simulink model "model"  (R2016a)
(part 4 of 4)

  220_kV_Połaniec___Chmielów_CN_199098053_220000_CN_191352746_220000/RConn1 -- "T_199098053_400000;220000;110000;15000_Stacja_elektroenergetyczna_\"Połaniec\"_400_220_110kV"/RConn1 -- 220_kV_Połaniec___Radkowice_CN_199098053_220000_CN_199098055_220000/RConn1 -- _CN_199098053_220000_CN_130207099_220000/LConn1 -- L_199098053/LConn1
  220_kV_Połaniec___Chmielów_CN_199098053_220000_CN_191352746_220000/RConn2 -- "T_199098053_400000;220000;110000;15000_Stacja_elektroenergetyczna_\"Połaniec\"_400_220_110kV"/RConn2 -- 220_kV_Połaniec___Radkowice_CN_199098053_220000_CN_199098055_220000/RConn2 -- _CN_199098053_220000_CN_130207099_220000/LConn2 -- L_199098053/LConn2
  220_kV_Połaniec___Chmielów_CN_199098053_220000_CN_191352746_220000/RConn3 -- "T_199098053_400000;220000;110000;15000_Stacja_elektroenergetyczna_\"Połaniec\"_400_220_110kV"/RConn3 -- 220_kV_Połaniec___Radkowice_CN_199098053_220000_CN_199098055_220000/RConn3 -- _CN_199098053_220000_CN_130207099_220000/LConn3 -- L_199098053/LConn3 -- bus86/LConn1
  _CN_199098053_220000_CN_130207099_220000/RConn1 -- G_130207099_Elektrownia_Połaniec/RConn1 -- _CN_199098053_400000_CN_130207099_220000/LConn1
  _CN_199098053_220000_CN_130207099_220000/RConn2 -- G_130207099_Elektrownia_Połaniec/RConn2 -- _CN_199098053_400000_CN_130207099_220000/LConn2
  _CN_199098053_220000_CN_130207099_220000/RConn3 -- G_130207099_Elektrownia_Połaniec/RConn3 -- _CN_199098053_400000_CN_130207099_220000/LConn3 -- bus87/LConn1
  _CN_254235846_220000_CN_189851841_220000/RConn1 -- "T_254235846_400000;110000_Stacja_elektroenergetyczna_\"Ostrowiec\"_400_110_kV"/RConn1 -- L_254235846/LConn1
  _CN_254235846_220000_CN_189851841_220000/RConn2 -- "T_254235846_400000;110000_Stacja_elektroenergetyczna_\"Ostrowiec\"_400_110_kV"/RConn2 -- L_254235846/LConn2
  _CN_254235846_220000_CN_189851841_220000/RConn3 -- "T_254235846_400000;110000_Stacja_elektroenergetyczna_\"Ostrowiec\"_400_110_kV"/RConn3 -- L_254235846/LConn3 -- bus88/LConn1
  T_179279860_220000;110000_Stacja_elektroenergetyczna_„Ząbkowice”_220_110_kV/LConn1 -- 220kV_Ząbkowice___Groszowice_CN_336990960_220000_CN_179279860_220000/RConn1
  T_179279860_220000;110000_Stacja_elektroenergetyczna_„Ząbkowice”_220_110_kV/LConn2 -- 220kV_Ząbkowice___Groszowice_CN_336990960_220000_CN_179279860_220000/RConn2
  220kV_Ząbkowice___Groszowice_CN_336990960_220000_CN_179279860_220000/RConn3 -- T_179279860_220000;110000_Stacja_elektroenergetyczna_„Ząbkowice”_220_110_kV/LConn3 -- bus89/LConn1
  220kV_Turów___Mikułowa_CN_111615226_220000_CN_90038401_220000/RConn1 -- G_90038401_Elektrownia_Turów/RConn1 -- 400kV_Turów___Mikułowa_CN_111615226_400000_CN_90038401_220000/LConn1
  220kV_Turów___Mikułowa_CN_111615226_220000_CN_90038401_220000/RConn2 -- G_90038401_Elektrownia_Turów/RConn2 -- 400kV_Turów___Mikułowa_CN_111615226_400000_CN_90038401_220000/LConn2
  220kV_Turów___Mikułowa_CN_111615226_220000_CN_90038401_220000/RConn3 -- G_90038401_Elektrownia_Turów/RConn3 -- 400kV_Turów___Mikułowa_CN_111615226_400000_CN_90038401_220000/LConn3 -- bus90/LConn1
  220kV_Joachimów___Huta_Częstochowa_CN_224727316_220000_CN_217899005_220000/LConn1 -- "T_224727316__Stacja_elektroenergetyczna_\"Huta_Częstochowa\"_220_110_kV"/LConn1 -- 220kV_Joachimów___Huta_Częstochowa_CN_224727316_220000_CN_66161634_220000/RConn1 -- 220kV_Joachimów___Huta_Częstochowa_CN_224727316_220000_CN_241842600_220000/RConn1
  220kV_Joachimów___Huta_Częstochowa_CN_224727316_220000_CN_217899005_220000/LConn2 -- "T_224727316__Stacja_elektroenergetyczna_\"Huta_Częstochowa\"_220_110_kV"/LConn2 -- 220kV_Joachimów___Huta_Częstochowa_CN_224727316_220000_CN_66161634_220000/RConn2 -- 220kV_Joachimów___Huta_Częstochowa_CN_224727316_220000_CN_241842600_220000/RConn2
  220kV_Joachimów___Huta_Częstochowa_CN_224727316_220000_CN_217899005_220000/LConn3 -- "T_224727316__Stacja_elektroenergetyczna_\"Huta_Częstochowa\"_220_110_kV"/LConn3 -- 220kV_Joachimów___Huta_Częstochowa_CN_224727316_220000_CN_66161634_220000/RConn3 -- 220kV_Joachimów___Huta_Częstochowa_CN_224727316_220000_CN_241842600_220000/RConn3 -- bus91/LConn1
  "T_217899005_220000;110000_Stacja_elektroenergetyczna_\"Wrzosowa\"_220_110_kV"/LConn1 -- 220kV_Joachimów___Huta_Częstochowa_CN_224727316_220000_CN_217899005_220000/RConn1
  "T_217899005_220000;110000_Stacja_elektroenergetyczna_\"Wrzosowa\"_220_110_kV"/LConn2 -- 220kV_Joachimów___Huta_Częstochowa_CN_224727316_220000_CN_217899005_220000/RConn2
  220kV_Joachimów___Huta_Częstochowa_CN_224727316_220000_CN_217899005_220000/RConn3 -- "T_217899005_220000;110000_Stacja_elektroenergetyczna_\"Wrzosowa\"_220_110_kV"/LConn3 -- bus92/LConn1
  220_kV_Dunowo___Żydowo_CN_178838661_220000_CN_175406958_220000/RConn1 -- "T_175406958_400000;220000;110000_Stacja_elektroenergetyczna_\"Dunowo\"_400_220_110_kV"/RConn1 -- L_175406958/LConn1
  220_kV_Dunowo___Żydowo_CN_178838661_220000_CN_175406958_220000/RConn2 -- "T_175406958_400000;220000;110000_Stacja_elektroenergetyczna_\"Dunowo\"_400_220_110_kV"/RConn2 -- L_175406958/LConn2
  220_kV_Dunowo___Żydowo_CN_178838661_220000_CN_175406958_220000/RConn3 -- "T_175406958_400000;220000;110000_Stacja_elektroenergetyczna_\"Dunowo\"_400_220_110_kV"/RConn3 -- L_175406958/LConn3 -- bus93/LConn1
  T_29098336_220000;110000_Stacja_elektroenergetyczna_„Piaseczno”_220_110_kV/LConn1 -- 220kV_Mory___Piaseczno_CN_29115701_220000_CN_29098336_220000/RConn1
  T_29098336_220000;110000_Stacja_elektroenergetyczna_„Piaseczno”_220_110_kV/LConn2 -- 220kV_Mory___Piaseczno_CN_29115701_220000_CN_29098336_220000/RConn2
  220kV_Mory___Piaseczno_CN_29115701_220000_CN_29098336_220000/RConn3 -- T_29098336_220000;110000_Stacja_elektroenergetyczna_„Piaseczno”_220_110_kV/LConn3 -- bus94/LConn1
  "T_255293400_220000;110000_Stacja_elektroenergetyczna_\"Bydgoszcz_Zachód\"_220_110_kV"/LConn1 -- 220kV_Jasiniec___Bydgoszcz_Zachód_CN_46235456_220000_CN_255293400_220000/RConn1
  "T_255293400_220000;110000_Stacja_elektroenergetyczna_\"Bydgoszcz_Zachód\"_220_110_kV"/LConn2 -- 220kV_Jasiniec___Bydgoszcz_Zachód_CN_46235456_220000_CN_255293400_220000/RConn2
  220kV_Jasiniec___Bydgoszcz_Zachód_CN_46235456_220000_CN_255293400_220000/RConn3 -- "T_255293400_220000;110000_Stacja_elektroenergetyczna_\"Bydgoszcz_Zachód\"_220_110_kV"/LConn3 -- bus95/LConn1
  220kV_Mokre___Chełm_CN_194903381_220000_CN_170368942_220000/RConn1 -- "T_194903381_220000;110000_Stacja_elektroenergetyczna_\"Chełm\"_220_110_kV"/LConn1 -- 220kV_Mokre___Chełm_CN_194903381_220000_CN_170249563_220000/RConn1
  220kV_Mokre___Chełm_CN_194903381_220000_CN_170368942_220000/RConn2 -- "T_194903381_220000;110000_Stacja_elektroenergetyczna_\"Chełm\"_220_110_kV"/LConn2 -- 220kV_Mokre___Chełm_CN_194903381_220000_CN_170249563_220000/RConn2
  220kV_Mokre___Chełm_CN_194903381_220000_CN_170368942_220000/RConn3 -- "T_194903381_220000;110000_Stacja_elektroenergetyczna_\"Chełm\"_220_110_kV"/LConn3 -- 220kV_Mokre___Chełm_CN_194903381_220000_CN_170249563_220000/RConn3 -- bus96/LConn1
  "G_221120858_Elektrociepłownia_\"Zielona_Góra\"_S_A_"/RConn1 -- 220kV_Leśniów___Zielona_Góra_CN_158232924_220000_CN_221120858_220000/RConn1
  "G_221120858_Elektrociepłownia_\"Zielona_Góra\"_S_A_"/RConn2 -- 220kV_Leśniów___Zielona_Góra_CN_158232924_220000_CN_221120858_220000/RConn2
  220kV_Leśniów___Zielona_Góra_CN_158232924_220000_CN_221120858_220000/RConn3 -- "G_221120858_Elektrociepłownia_\"Zielona_Góra\"_S_A_"/RConn3 -- bus97/LConn1
  _CN_39428977_220000_CN_35222596_220000/RConn1 -- G_35222596_Elektrownia_Dolna_Odra/RConn1 -- _CN_39428977_400000_CN_35222596_220000/LConn1
  _CN_39428977_220000_CN_35222596_220000/RConn2 -- G_35222596_Elektrownia_Dolna_Odra/RConn2 -- _CN_39428977_400000_CN_35222596_220000/LConn2
  _CN_39428977_220000_CN_35222596_220000/RConn3 -- G_35222596_Elektrownia_Dolna_Odra/RConn3 -- _CN_39428977_400000_CN_35222596_220000/LConn3 -- bus98/LConn1
  T_177493901__/LConn1 -- _CN_39428977_220000_CN_177493901_220000/RConn1
  T_177493901__/LConn2 -- _CN_39428977_220000_CN_177493901_220000/RConn2
  _CN_39428977_220000_CN_177493901_220000/RConn3 -- T_177493901__/LConn3 -- bus99/LConn1
  T_240806770__/LConn1 -- _CN_240806770_220000_CN_153838553_220000/RConn1
  T_240806770__/LConn2 -- _CN_240806770_220000_CN_153838553_220000/RConn2
  _CN_240806770_220000_CN_153838553_220000/RConn3 -- T_240806770__/LConn3 -- bus100/LConn1
  _CN_179138441_220000_CN_276291999_220000/RConn1 -- "T_276291999__Stacja_elektroenergetyczna_\"Świebodzice\"_400_kV"/RConn1 -- L_276291999/LConn1
  _CN_179138441_220000_CN_276291999_220000/RConn2 -- "T_276291999__Stacja_elektroenergetyczna_\"Świebodzice\"_400_kV"/RConn2 -- L_276291999/LConn2
  _CN_179138441_220000_CN_276291999_220000/RConn3 -- "T_276291999__Stacja_elektroenergetyczna_\"Świebodzice\"_400_kV"/RConn3 -- L_276291999/LConn3 -- bus101/LConn1
  "T_198635989_220000;110000;30000;15000_Stacja_elektroenergetyczna_\"Boguchwała\"_220_110_kV"/LConn1 -- 220_kV_Chmielów___Boguchwała_CN_191352746_220000_CN_198635989_220000/RConn1
  "T_198635989_220000;110000;30000;15000_Stacja_elektroenergetyczna_\"Boguchwała\"_220_110_kV"/LConn2 -- 220_kV_Chmielów___Boguchwała_CN_191352746_220000_CN_198635989_220000/RConn2
  220_kV_Chmielów___Boguchwała_CN_191352746_220000_CN_198635989_220000/RConn3 -- "T_198635989_220000;110000;30000;15000_Stacja_elektroenergetyczna_\"Boguchwała\"_220_110_kV"/LConn3 -- bus102/LConn1
  400kV_Dobrzeń___Pasikurowice_CN_255277953_400000_CN_79033485_400000/LConn1 -- "T_255277953_400000;110000_Stacja_elektroenergetyczna_\"Dobrzeń\"_400_110_kV"/LConn1 -- 400kV_Dobrzeń___Pasikurowice_CN_255277953_400000_CN_171917072_400000/LConn1 -- 400kV_Dobrzeń___Pasikurowice_CN_255277953_400000_CN_241842600_400000/LConn1 -- 400kV_Dobrzeń___Wielopole_CN_255277953_400000_CN_139452056_400000/LConn1
  400kV_Dobrzeń___Pasikurowice_CN_255277953_400000_CN_79033485_400000/LConn2 -- "T_255277953_400000;110000_Stacja_elektroenergetyczna_\"Dobrzeń\"_400_110_kV"/LConn2 -- 400kV_Dobrzeń___Pasikurowice_CN_255277953_400000_CN_171917072_400000/LConn2 -- 400kV_Dobrzeń___Pasikurowice_CN_255277953_400000_CN_241842600_400000/LConn2 -- 400kV_Dobrzeń___Wielopole_CN_255277953_400000_CN_139452056_400000/LConn2
  400kV_Dobrzeń___Pasikurowice_CN_255277953_400000_CN_79033485_400000/LConn3 -- "T_255277953_400000;110000_Stacja_elektroenergetyczna_\"Dobrzeń\"_400_110_kV"/LConn3 -- 400kV_Dobrzeń___Pasikurowice_CN_255277953_400000_CN_171917072_400000/LConn3 -- 400kV_Dobrzeń___Pasikurowice_CN_255277953_400000_CN_241842600_400000/LConn3 -- 400kV_Dobrzeń___Wielopole_CN_255277953_400000_CN_139452056_400000/LConn3 -- bus103/LConn1
  400kV_Dobrzeń___Pasikurowice_CN_255277953_400000_CN_79033485_400000/RConn1 -- T_79033485_400000;110000_Stacja_elektroenergetyczna_„Pasikurowice”_400_110_kV/LConn1 -- 400kV_Pasikurowice___Ostrów_CN_79033485_400000_CN_255293403_400000/LConn1 -- 400kV_Pasikurowice___Wrocław_CN_79033485_400000_CN_154510504_400000/LConn1 -- 400kV_Czarna___Pasikurowice_CN_79033485_400000_CN_154894455_400000/LConn1
  400kV_Dobrzeń___Pasikurowice_CN_255277953_400000_CN_79033485_400000/RConn2 -- T_79033485_400000;110000_Stacja_elektroenergetyczna_„Pasikurowice”_400_110_kV/LConn2 -- 400kV_Pasikurowice___Ostrów_CN_79033485_400000_CN_255293403_400000/LConn2 -- 400kV_Pasikurowice___Wrocław_CN_79033485_400000_CN_154510504_400000/LConn2 -- 400kV_Czarna___Pasikurowice_CN_79033485_400000_CN_154894455_400000/LConn2
  400kV_Dobrzeń___Pasikurowice_CN_255277953_400000_CN_79033485_400000/RConn3 -- T_79033485_400000;110000_Stacja_elektroenergetyczna_„Pasikurowice”_400_110_kV/LConn3 -- 400kV_Pasikurowice___Ostrów_CN_79033485_400000_CN_255293403_400000/LConn3 -- 400kV_Pasikurowice___Wrocław_CN_79033485_400000_CN_154510504_400000/LConn3 -- bus104/LConn1 -- 400kV_Czarna___Pasikurowice_CN_79033485_400000_CN_154894455_400000/LConn3
  400kV_Dobrzeń___Pasikurowice_CN_255277953_400000_CN_171917072_400000/RConn1 -- T_171917072_400000;110000_Stacja_elektroenergetyczna_„Trębaczew”_400_110_kV/LConn1 -- 400kV_Rogowiec___Trębaczew_CN_171917072_400000_CN_255293403_400000/LConn1 -- 400kV_Rogowiec___Trębaczew_CN_171917072_400000_CN_293484891_400000/LConn1
  400kV_Dobrzeń___Pasikurowice_CN_255277953_400000_CN_171917072_400000/RConn2 -- T_171917072_400000;110000_Stacja_elektroenergetyczna_„Trębaczew”_400_110_kV/LConn2 -- 400kV_Rogowiec___Trębaczew_CN_171917072_400000_CN_255293403_400000/LConn2 -- 400kV_Rogowiec___Trębaczew_CN_171917072_400000_CN_293484891_400000/LConn2
  400kV_Dobrzeń___Pasikurowice_CN_255277953_400000_CN_171917072_400000/RConn3 -- T_171917072_400000;110000_Stacja_elektroenergetyczna_„Trębaczew”_400_110_kV/LConn3 -- 400kV_Rogowiec___Trębaczew_CN_171917072_400000_CN_255293403_400000/LConn3 -- 400kV_Rogowiec___Trębaczew_CN_171917072_400000_CN_293484891_400000/LConn3 -- bus105/LConn1
  400kV_Dobrzeń___Pasikurowice_CN_255277953_400000_CN_241842600_400000/RConn1 -- T_241842600_400000;220000_Stacja_elektroenergetyczna_„Joachimów”_400_220_kV/LConn1 -- 400kV_Wielopole___Joachimów_CN_241842600_400000_CN_40946784_400000/LConn1 -- 400kV_Wielopole___Joachimów_CN_241842600_400000_CN_66161634_400000/LConn1 -- 400kV_Wielopole___Joachimów_CN_241842600_400000_CN_293489607_400000/LConn1 -- 400kV_Wielopole___Joachimów_CN_241842600_400000_CN_139452056_400000/LConn1 -- 400kV_Wielopole___Joachimów_CN_241842600_400000_CN_293484891_400000/LConn1
  400kV_Dobrzeń___Pasikurowice_CN_255277953_400000_CN_241842600_400000/RConn2 -- T_241842600_400000;220000_Stacja_elektroenergetyczna_„Joachimów”_400_220_kV/LConn2 -- 400kV_Wielopole___Joachimów_CN_241842600_400000_CN_40946784_400000/LConn2 -- 400kV_Wielopole___Joachimów_CN_241842600_400000_CN_66161634_400000/LConn2 -- 400kV_Wielopole___Joachimów_CN_241842600_400000_CN_293489607_400000/LConn2 -- 400kV_Wielopole___Joachimów_CN_241842600_400000_CN_139452056_400000/LConn2 -- 400kV_Wielopole___Joachimów_CN_241842600_400000_CN_293484891_400000/LConn2
  400kV_Dobrzeń___Pasikurowice_CN_255277953_400000_CN_241842600_400000/RConn3 -- T_241842600_400000;220000_Stacja_elektroenergetyczna_„Joachimów”_400_220_kV/LConn3 -- 400kV_Wielopole___Joachimów_CN_241842600_400000_CN_40946784_400000/LConn3 -- 400kV_Wielopole___Joachimów_CN_241842600_400000_CN_66161634_400000/LConn3 -- 400kV_Wielopole___Joachimów_CN_241842600_400000_CN_293489607_400000/LConn3 -- 400kV_Wielopole___Joachimów_CN_241842600_400000_CN_139452056_400000/LConn3 -- 400kV_Wielopole___Joachimów_CN_241842600_400000_CN_293484891_400000/LConn3 -- bus106/LConn1
  400kV_Dobrzeń___Wielopole_CN_255277953_400000_CN_139452056_400000/RConn1 -- T_139452056_400000;220000;110000_Stacja_elektroenergetyczna_„Wielopole”_400_220_110_kV/LConn1 -- 400kV_Wielopole___Joachimów_CN_241842600_400000_CN_139452056_400000/RConn1
  400kV_Dobrzeń___Wielopole_CN_255277953_400000_CN_139452056_400000/RConn2 -- T_139452056_400000;220000;110000_Stacja_elektroenergetyczna_„Wielopole”_400_220_110_kV/LConn2 -- 400kV_Wielopole___Joachimów_CN_241842600_400000_CN_139452056_400000/RConn2
  400kV_Dobrzeń___Wielopole_CN_255277953_400000_CN_139452056_400000/RConn3 -- T_139452056_400000;220000;110000_Stacja_elektroenergetyczna_„Wielopole”_400_220_110_kV/LConn3 -- 400kV_Wielopole___Joachimów_CN_241842600_400000_CN_139452056_400000/RConn3 -- bus107/LConn1
  400kV_Wielopole___Joachimów_CN_241842600_400000_CN_40946784_400000/RConn1 -- T_40946784_400000;110000_Stacja_elektroenergetyczna_„Tucznawa”_400_110_kV/LConn1 -- 400_kV_Tarnów___Krosno_Iskrzynia_CN_166838338_400000_CN_40946784_400000/LConn1
  400kV_Wielopole___Joachimów_CN_241842600_400000_CN_40946784_400000/RConn2 -- T_40946784_400000;110000_Stacja_elektroenergetyczna_„Tucznawa”_400_110_kV/LConn2 -- 400_kV_Tarnów___Krosno_Iskrzynia_CN_166838338_400000_CN_40946784_400000/LConn2
  400kV_Wielopole___Joachimów_CN_241842600_400000_CN_40946784_400000/RConn3 -- T_40946784_400000;110000_Stacja_elektroenergetyczna_„Tucznawa”_400_110_kV/LConn3 -- 400_kV_Tarnów___Krosno_Iskrzynia_CN_166838338_400000_CN_40946784_400000/LConn3 -- bus108/LConn1
  "T_66161634_400000;220000;110000_Stacja_elektroenergetyczna_\"Łagisza\"_400_220_110_kV"/LConn1 -- 400kV_Wielopole___Joachimów_CN_241842600_400000_CN_66161634_400000/RConn1
  "T_66161634_400000;220000;110000_Stacja_elektroenergetyczna_\"Łagisza\"_400_220_110_kV"/LConn2 -- 400kV_Wielopole___Joachimów_CN_241842600_400000_CN_66161634_400000/RConn2
  400kV_Wielopole___Joachimów_CN_241842600_400000_CN_66161634_400000/RConn3 -- "T_66161634_400000;220000;110000_Stacja_elektroenergetyczna_\"Łagisza\"_400_220_110_kV"/LConn3 -- bus109/LConn1
  "T_293489607_400000;110000_Stacja_elektroenergetyczna_\"Rokitnica\"_400_110kV"/LConn1 -- 400kV_Wielopole___Joachimów_CN_241842600_400000_CN_293489607_400000/RConn1
  "T_293489607_400000;110000_Stacja_elektroenergetyczna_\"Rokitnica\"_400_110kV"/LConn2 -- 400kV_Wielopole___Joachimów_CN_241842600_400000_CN_293489607_400000/RConn2
  400kV_Wielopole___Joachimów_CN_241842600_400000_CN_293489607_400000/RConn3 -- "T_293489607_400000;110000_Stacja_elektroenergetyczna_\"Rokitnica\"_400_110kV"/LConn3 -- bus110/LConn1
  400kV_Wielopole___Joachimów_CN_241842600_400000_CN_293484891_400000/RConn1 -- "T_293484891_400000;220000_Stacja_elektroenergetyczna_\"Rogowiec\"_400_220_kV"/LConn1 -- 400kV_Rogowiec___Trębaczew_CN_171917072_400000_CN_293484891_400000/RConn1 -- 400kV_Rogowiec___Płock_CN_144646702_400000_CN_293484891_400000/LConn1
  400kV_Wielopole___Joachimów_CN_241842600_400000_CN_293484891_400000/RConn2 -- "T_293484891_400000;220000_Stacja_elektroenergetyczna_\"Rogowiec\"_400_220_kV"/LConn2 -- 400kV_Rogowiec___Trębaczew_CN_171917072_400000_CN_293484891_400000/RConn2 -- 400kV_Rogowiec___Płock_CN_144646702_400000_CN_293484891_400000/LConn2
  400kV_Wielopole___Joachimów_CN_241842600_400000_CN_293484891_400000/RConn3 -- "T_293484891_400000;220000_Stacja_elektroenergetyczna_\"Rogowiec\"_400_220_kV"/LConn3 -- 400kV_Rogowiec___Trębaczew_CN_171917072_400000_CN_293484891_400000/RConn3 -- 400kV_Rogowiec___Płock_CN_144646702_400000_CN_293484891_400000/LConn3 -- bus111/LConn1
  400kV_Plewiska___Ostrów_CN_32036484_400000_CN_254938713_400000/LConn1 -- "T_32036484_400000;220000;110000_Stacja_elektroenergetyczna_\"Plewiska\"_400_220_110_kV"/LConn1 -- 400kV_Krajnik___Plewiska_CN_32036484_400000_CN_39428977_400000/LConn1
  400kV_Plewiska___Ostrów_CN_32036484_400000_CN_254938713_400000/LConn2 -- "T_32036484_400000;220000;110000_Stacja_elektroenergetyczna_\"Plewiska\"_400_220_110_kV"/LConn2 -- 400kV_Krajnik___Plewiska_CN_32036484_400000_CN_39428977_400000/LConn2
  400kV_Plewiska___Ostrów_CN_32036484_400000_CN_254938713_400000/LConn3 -- "T_32036484_400000;220000;110000_Stacja_elektroenergetyczna_\"Plewiska\"_400_220_110_kV"/LConn3 -- 400kV_Krajnik___Plewiska_CN_32036484_400000_CN_39428977_400000/LConn3 -- bus112/LConn1
  400kV_Plewiska___Ostrów_CN_32036484_400000_CN_254938713_400000/RConn1 -- T_254938713_400000;110000_Stacja_elektroenergetyczna_Kromolice_400_110kV/LConn1 -- 400kV_Kromolice___Ostrów_+_110kV_Kromolice___Środa_CN_254938713_400000_CN_255293403_400000/LConn1
  400kV_Plewiska___Ostrów_CN_32036484_400000_CN_254938713_400000/RConn2 -- T_254938713_400000;110000_Stacja_elektroenergetyczna_Kromolice_400_110kV/LConn2 -- 400kV_Kromolice___Ostrów_+_110kV_Kromolice___Środa_CN_254938713_400000_CN_255293403_400000/LConn2
  400kV_Plewiska___Ostrów_CN_32036484_400000_CN_254938713_400000/RConn3 -- T_254938713_400000;110000_Stacja_elektroenergetyczna_Kromolice_400_110kV/LConn3 -- 400kV_Kromolice___Ostrów_+_110kV_Kromolice___Środa_CN_254938713_400000_CN_255293403_400000/LConn3 -- bus113/LConn1
  400kV_Krajnik___Plewiska_CN_32036484_400000_CN_39428977_400000/RConn1 -- "T_39428977_400000;220000_Stacja_elektroenergetyczna_\"Krajnik\"_400_220_kV"/LConn1 -- _CN_39428977_400000_CN_35222596_220000/RConn1 -- 400kV_Krajnik___Morzyczyn_CN_32943179_400000_CN_39428977_400000/LConn1
  400kV_Krajnik___Plewiska_CN_32036484_400000_CN_39428977_400000/RConn2 -- "T_39428977_400000;220000_Stacja_elektroenergetyczna_\"Krajnik\"_400_220_kV"/LConn2 -- _CN_39428977_400000_CN_35222596_220000/RConn2 -- 400kV_Krajnik___Morzyczyn_CN_32943179_400000_CN_39428977_400000/LConn2
  400kV_Krajnik___Plewiska_CN_32036484_400000_CN_39428977_400000/RConn3 -- "T_39428977_400000;220000_Stacja_elektroenergetyczna_\"Krajnik\"_400_220_kV"/LConn3 -- _CN_39428977_400000_CN_35222596_220000/RConn3 -- bus114/LConn1 -- 400kV_Krajnik___Morzyczyn_CN_32943179_400000_CN_39428977_400000/LConn3
  T_169979525__/LConn1 -- _CN_169979525_400000_CN_255314292_400000/LConn1
  T_169979525__/LConn2 -- _CN_169979525_400000_CN_255314292_400000/LConn2
  _CN_169979525_400000_CN_255314292_400000/LConn3 -- T_169979525__/LConn3 -- bus115/LConn1
  _CN_169979525_400000_CN_255314292_400000/RConn1 -- T_255314292_450000;400000_SwePol_HVDC_Static_Inverter_Plant/LConn1 -- _CN_169979526_400000_CN_255314292_400000/LConn1 -- _CN_169979527_400000_CN_255314292_400000/LConn1 -- _CN_169979538_400000_CN_255314292_400000/LConn1 -- _CN_255314292_400000_CN_365677253_400000/LConn1
  _CN_169979525_400000_CN_255314292_400000/RConn2 -- T_255314292_450000;400000_SwePol_HVDC_Static_Inverter_Plant/LConn2 -- _CN_169979526_400000_CN_255314292_400000/LConn2 -- _CN_169979527_400000_CN_255314292_400000/LConn2 -- _CN_169979538_400000_CN_255314292_400000/LConn2 -- _CN_255314292_400000_CN_365677253_400000/LConn2
  _CN_169979525_400000_CN_255314292_400000/RConn3 -- T_255314292_450000;400000_SwePol_HVDC_Static_Inverter_Plant/LConn3 -- _CN_169979526_400000_CN_255314292_400000/LConn3 -- _CN_169979527_400000_CN_255314292_400000/LConn3 -- _CN_169979538_400000_CN_255314292_400000/LConn3 -- _CN_255314292_400000_CN_365677253_400000/LConn3 -- bus116/LConn1
  T_169979526__Capacitator_Bank/LConn1 -- _CN_169979526_400000_CN_255314292_400000/RConn1
  T_169979526__Capacitator_Bank/LConn2 -- _CN_169979526_400000_CN_255314292_400000/RConn2
  _CN_169979526_400000_CN_255314292_400000/RConn3 -- T_169979526__Capacitator_Bank/LConn3 -- bus117/LConn1
  T_169979527__Harmonic_Filter/LConn1 -- _CN_169979527_400000_CN_255314292_400000/RConn1
  T_169979527__Harmonic_Filter/LConn2 -- _CN_169979527_400000_CN_255314292_400000/RConn2
  _CN_169979527_400000_CN_255314292_400000/RConn3 -- T_169979527__Harmonic_Filter/LConn3 -- bus118/LConn1
  400kV_Grudziądz_Węgrowo___Płock_CN_46092396_400000_CN_144646702_400000/LConn1 -- "T_46092396_400000;220000;110000_Stacja_elektroenergetyczna_\"Grudziądz___Węgrowo\"_400_220_110_kV"/LConn1 -- 400kV_Grudziądz_Węgrowo___Gdańsk_Błonia_CN_46092396_400000_CN_112614319_400000/LConn1
  400kV_Grudziądz_Węgrowo___Płock_CN_46092396_400000_CN_144646702_400000/LConn2 -- "T_46092396_400000;220000;110000_Stacja_elektroenergetyczna_\"Grudziądz___Węgrowo\"_400_220_110_kV"/LConn2 -- 400kV_Grudziądz_Węgrowo___Gdańsk_Błonia_CN_46092396_400000_CN_112614319_400000/LConn2
  400kV_Grudziądz_Węgrowo___Płock_CN_46092396_400000_CN_144646702_400000/LConn3 -- "T_46092396_400000;220000;110000_Stacja_elektroenergetyczna_\"Grudziądz___Węgrowo\"_400_220_110_kV"/LConn3 -- 400kV_Grudziądz_Węgrowo___Gdańsk_Błonia_CN_46092396_400000_CN_112614319_400000/LConn3 -- bus119/LConn1
  400kV_Grudziądz_Węgrowo___Płock_CN_46092396_400000_CN_144646702_400000/RConn1 -- T_144646702_400000;110000_Stacja_elektroenergetyczna_„Płock”_400_110_kV/LConn1 -- 400kV_Rogowiec___Płock_CN_144646702_400000_CN_251239544_400000/LConn1 -- 400kV_Rogowiec___Płock_CN_144646702_400000_CN_293484891_400000/RConn1
  400kV_Grudziądz_Węgrowo___Płock_CN_46092396_400000_CN_144646702_400000/RConn2 -- T_144646702_400000;110000_Stacja_elektroenergetyczna_„Płock”_400_110_kV/LConn2 -- 400kV_Rogowiec___Płock_CN_144646702_400000_CN_251239544_400000/LConn2 -- 400kV_Rogowiec___Płock_CN_144646702_400000_CN_293484891_400000/RConn2
  400kV_Grudziądz_Węgrowo___Płock_CN_46092396_400000_CN_144646702_400000/RConn3 -- T_144646702_400000;110000_Stacja_elektroenergetyczna_„Płock”_400_110_kV/LConn3 -- 400kV_Rogowiec___Płock_CN_144646702_400000_CN_251239544_400000/LConn3 -- 400kV_Rogowiec___Płock_CN_144646702_400000_CN_293484891_400000/RConn3 -- bus120/LConn1
  400kV_Grudziądz_Węgrowo___Gdańsk_Błonia_CN_46092396_400000_CN_112614319_400000/RConn1 -- "T_112614319_400000;110000_Stacja_elektroenergetyczna_\"Gdańsk_Błonia\"_400_110_kV"/LConn1 -- 400kV_Gdańsk_Błonia___Olsztyn_Mątki_CN_101914781_400000_CN_112614319_400000/LConn1 -- 400kV_Gdańsk_Błonia___Żarnowiec_CN_86494356_400000_CN_112614319_400000/LConn1
  400kV_Grudziądz_Węgrowo___Gdańsk_Błonia_CN_46092396_400000_CN_112614319_400000/RConn2 -- "T_112614319_400000;110000_Stacja_elektroenergetyczna_\"Gdańsk_Błonia\"_400_110_kV"/LConn2 -- 400kV_Gdańsk_Błonia___Olsztyn_Mątki_CN_101914781_400000_CN_112614319_400000/LConn2 -- 400kV_Gdańsk_Błonia___Żarnowiec_CN_86494356_400000_CN_112614319_400000/LConn2
  400kV_Grudziądz_Węgrowo___Gdańsk_Błonia_CN_46092396_400000_CN_112614319_400000/RConn3 -- "T_112614319_400000;110000_Stacja_elektroenergetyczna_\"Gdańsk_Błonia\"_400_110_kV"/LConn3 -- 400kV_Gdańsk_Błonia___Olsztyn_Mątki_CN_101914781_400000_CN_112614319_400000/LConn3 -- bus121/LConn1 -- 400kV_Gdańsk_Błonia___Żarnowiec_CN_86494356_400000_CN_112614319_400000/LConn3
  400kV_Czarna___Pasikurowice_CN_79033485_400000_CN_154894455_400000/RConn1 -- "T_154894455_400000;110000_Stacja_elektroenergetyczna_\"Czarna\"_400_110_kV"/LConn1 -- 400kV_Mikułowa___Czarna_CN_154894455_400000_CN_111615226_400000/LConn1
  400kV_Czarna___Pasikurowice_CN_79033485_400000_CN_154894455_400000/RConn2 -- "T_154894455_400000;110000_Stacja_elektroenergetyczna_\"Czarna\"_400_110_kV"/LConn2 -- 400kV_Mikułowa___Czarna_CN_154894455_400000_CN_111615226_400000/LConn2
  400kV_Czarna___Pasikurowice_CN_79033485_400000_CN_154894455_400000/RConn3 -- "T_154894455_400000;110000_Stacja_elektroenergetyczna_\"Czarna\"_400_110_kV"/LConn3 -- 400kV_Mikułowa___Czarna_CN_154894455_400000_CN_111615226_400000/LConn3 -- bus122/LConn1
  400kV_Pasikurowice___Ostrów_CN_79033485_400000_CN_255293403_400000/RConn1 -- "T_255293403_400000;110000_Stacja_elektroenergetyczna_\"Ostrów\"_400_110_kV"/LConn1 -- 400kV_Rogowiec___Trębaczew_CN_171917072_400000_CN_255293403_400000/RConn1 -- 400kV_Kromolice___Ostrów_+_110kV_Kromolice___Środa_CN_254938713_400000_CN_255293403_400000/RConn1
  400kV_Pasikurowice___Ostrów_CN_79033485_400000_CN_255293403_400000/RConn2 -- "T_255293403_400000;110000_Stacja_elektroenergetyczna_\"Ostrów\"_400_110_kV"/LConn2 -- 400kV_Rogowiec___Trębaczew_CN_171917072_400000_CN_255293403_400000/RConn2 -- 400kV_Kromolice___Ostrów_+_110kV_Kromolice___Środa_CN_254938713_400000_CN_255293403_400000/RConn2
  400kV_Pasikurowice___Ostrów_CN_79033485_400000_CN_255293403_400000/RConn3 -- "T_255293403_400000;110000_Stacja_elektroenergetyczna_\"Ostrów\"_400_110_kV"/LConn3 -- 400kV_Rogowiec___Trębaczew_CN_171917072_400000_CN_255293403_400000/RConn3 -- 400kV_Kromolice___Ostrów_+_110kV_Kromolice___Środa_CN_254938713_400000_CN_255293403_400000/RConn3 -- bus123/LConn1
  400kV_Pasikurowice___Wrocław_CN_79033485_400000_CN_154510504_400000/RConn1 -- "T_154510504__Stacja_elektroenergetyczna_\"Wrocław\"_400_110kV"/LConn1 -- Świebodzice___Wrocław_CN_276291999_400000_CN_154510504_400000/LConn1
  400kV_Pasikurowice___Wrocław_CN_79033485_400000_CN_154510504_400000/RConn2 -- "T_154510504__Stacja_elektroenergetyczna_\"Wrocław\"_400_110kV"/LConn2 -- Świebodzice___Wrocław_CN_276291999_400000_CN_154510504_400000/LConn2
  400kV_Pasikurowice___Wrocław_CN_79033485_400000_CN_154510504_400000/RConn3 -- "T_154510504__Stacja_elektroenergetyczna_\"Wrocław\"_400_110kV"/LConn3 -- Świebodzice___Wrocław_CN_276291999_400000_CN_154510504_400000/LConn3 -- bus124/LConn1
  T_169979538__Capacitator_Bank/LConn1 -- _CN_169979538_400000_CN_255314292_400000/RConn1
  T_169979538__Capacitator_Bank/LConn2 -- _CN_169979538_400000_CN_255314292_400000/RConn2
  _CN_169979538_400000_CN_255314292_400000/RConn3 -- T_169979538__Capacitator_Bank/LConn3 -- bus125/LConn1
  400kV_Gdańsk_Błonia___Żarnowiec_CN_86494356_400000_CN_112614319_400000/RConn1 -- "T_86494356_400000;110000_Stacja_elektroenergetyczna_\"Żarnowiec\"_400_110_kV"/LConn1 -- 400kV_Gdańsk_Błonia___Żarnowiec_CN_86494356_400000_CN_154838041_400000/LConn1 -- _CN_86494356_400000_CN_53294547_400000/LConn1 -- 400kV_Słupsk___Żarnowiec_CN_86494356_400000_CN_305265212_400000/LConn1
  400kV_Gdańsk_Błonia___Żarnowiec_CN_86494356_400000_CN_112614319_400000/RConn2 -- "T_86494356_400000;110000_Stacja_elektroenergetyczna_\"Żarnowiec\"_400_110_kV"/LConn2 -- 400kV_Gdańsk_Błonia___Żarnowiec_CN_86494356_400000_CN_154838041_400000/LConn2 -- _CN_86494356_400000_CN_53294547_400000/LConn2 -- 400kV_Słupsk___Żarnowiec_CN_86494356_400000_CN_305265212_400000/LConn2
  400kV_Gdańsk_Błonia___Żarnowiec_CN_86494356_400000_CN_112614319_400000/RConn3 -- "T_86494356_400000;110000_Stacja_elektroenergetyczna_\"Żarnowiec\"_400_110_kV"/LConn3 -- 400kV_Gdańsk_Błonia___Żarnowiec_CN_86494356_400000_CN_154838041_400000/LConn3 -- _CN_86494356_400000_CN_53294547_400000/LConn3 -- 400kV_Słupsk___Żarnowiec_CN_86494356_400000_CN_305265212_400000/LConn3 -- bus126/LConn1
  "T_154838041_400000;220000;110000_Stacja_elektroenergetyczna_\"Gdańsk_I\"_400_220_110_kV"/LConn1 -- 400kV_Gdańsk_Błonia___Żarnowiec_CN_86494356_400000_CN_154838041_400000/RConn1
  "T_154838041_400000;220000;110000_Stacja_elektroenergetyczna_\"Gdańsk_I\"_400_220_110_kV"/LConn2 -- 400kV_Gdańsk_Błonia___Żarnowiec_CN_86494356_400000_CN_154838041_400000/RConn2
  400kV_Gdańsk_Błonia___Żarnowiec_CN_86494356_400000_CN_154838041_400000/RConn3 -- "T_154838041_400000;220000;110000_Stacja_elektroenergetyczna_\"Gdańsk_I\"_400_220_110_kV"/LConn3 -- bus127/LConn1
  G_53294547_Elektrownia_Wodna_Żarnowiec/RConn1 -- _CN_86494356_400000_CN_53294547_400000/RConn1
  G_53294547_Elektrownia_Wodna_Żarnowiec/RConn2 -- _CN_86494356_400000_CN_53294547_400000/RConn2
  _CN_86494356_400000_CN_53294547_400000/RConn3 -- G_53294547_Elektrownia_Wodna_Żarnowiec/RConn3 -- bus128/LConn1
  400kV_Słupsk___Żarnowiec_CN_86494356_400000_CN_305265212_400000/RConn1 -- "T_305265212_400000;110000_Stacja_elektrenergetyczna_400_110kV_\"Słupsk_Wierzbięcino\""/LConn1 -- system_1_CN_305265212_400000_CN_365677253_400000/LConn1
  400kV_Słupsk___Żarnowiec_CN_86494356_400000_CN_305265212_400000/RConn2 -- "T_305265212_400000;110000_Stacja_elektrenergetyczna_400_110kV_\"Słupsk_Wierzbięcino\""/LConn2 -- system_1_CN_305265212_400000_CN_365677253_400000/LConn2
  400kV_Słupsk___Żarnowiec_CN_86494356_400000_CN_305265212_400000/RConn3 -- "T_305265212_400000;110000_Stacja_elektrenergetyczna_400_110kV_\"Słupsk_Wierzbięcino\""/LConn3 -- system_1_CN_305265212_400000_CN_365677253_400000/LConn3 -- bus129/LConn1
  400kV_Słupsk___Dunowo_CN_175406958_400000_CN_365677253_400000/LConn1 -- "T_175406958_400000;220000;110000_Stacja_elektroenergetyczna_\"Dunowo\"_400_220_110_kV"/LConn1 -- _CN_175406958_400000_CN_216446549_400000/LConn1 -- 400kV_Morzyczyn___Dunowo_CN_175406958_400000_CN_32943179_400000/LConn1
  400kV_Słupsk___Dunowo_CN_175406958_400000_CN_365677253_400000/LConn2 -- "T_175406958_400000;220000;110000_Stacja_elektroenergetyczna_\"Dunowo\"_400_220_110_kV"/LConn2 -- _CN_175406958_400000_CN_216446549_400000/LConn2 -- 400kV_Morzyczyn___Dunowo_CN_175406958_400000_CN_32943179_400000/LConn2
  400kV_Słupsk___Dunowo_CN_175406958_400000_CN_365677253_400000/LConn3 -- "T_175406958_400000;220000;110000_Stacja_elektroenergetyczna_\"Dunowo\"_400_220_110_kV"/LConn3 -- _CN_175406958_400000_CN_216446549_400000/LConn3 -- bus130/LConn1 -- 400kV_Morzyczyn___Dunowo_CN_175406958_400000_CN_32943179_400000/LConn3
  400kV_Słupsk___Dunowo_CN_175406958_400000_CN_365677253_400000/RConn1 -- "T_365677253_400000;110000_Stacja_elektrenergetyczna_400_110kV_\"Słupsk_Wierzbięcino\""/LConn1 -- _CN_255314292_400000_CN_365677253_400000/RConn1 -- system_1_CN_305265212_400000_CN_365677253_400000/RConn1
  400kV_Słupsk___Dunowo_CN_175406958_400000_CN_365677253_400000/RConn2 -- "T_365677253_400000;110000_Stacja_elektrenergetyczna_400_110kV_\"Słupsk_Wierzbięcino\""/LConn2 -- _CN_255314292_400000_CN_365677253_400000/RConn2 -- system_1_CN_305265212_400000_CN_365677253_400000/RConn2
  400kV_Słupsk___Dunowo_CN_175406958_400000_CN_365677253_400000/RConn3 -- "T_365677253_400000;110000_Stacja_elektrenergetyczna_400_110kV_\"Słupsk_Wierzbięcino\""/LConn3 -- _CN_255314292_400000_CN_365677253_400000/RConn3 -- system_1_CN_305265212_400000_CN_365677253_400000/RConn3 -- bus131/LConn1
  400kV_Morzyczyn___Dunowo_CN_175406958_400000_CN_32943179_400000/RConn1 -- "T_32943179_400000;220000;110000_Stacja_elektroenergetyczna_\"Morzyczyn\"_400_220_110_kV"/LConn1 -- 400kV_Krajnik___Morzyczyn_CN_32943179_400000_CN_39428977_400000/RConn1
  400kV_Morzyczyn___Dunowo_CN_175406958_400000_CN_32943179_400000/RConn2 -- "T_32943179_400000;220000;110000_Stacja_elektroenergetyczna_\"Morzyczyn\"_400_220_110_kV"/LConn2 -- 400kV_Krajnik___Morzyczyn_CN_32943179_400000_CN_39428977_400000/RConn2
  400kV_Morzyczyn___Dunowo_CN_175406958_400000_CN_32943179_400000/RConn3 -- "T_32943179_400000;220000;110000_Stacja_elektroenergetyczna_\"Morzyczyn\"_400_220_110_kV"/LConn3 -- 400kV_Krajnik___Morzyczyn_CN_32943179_400000_CN_39428977_400000/RConn3 -- bus132/LConn1
  T_216446549__/LConn1 -- _CN_175406958_400000_CN_216446549_400000/RConn1
  T_216446549__/LConn2 -- _CN_175406958_400000_CN_216446549_400000/RConn2
  _CN_175406958_400000_CN_216446549_400000/RConn3 -- T_216446549__/LConn3 -- bus133/LConn1
  400kV_Kozienice___Miłosna_CN_99593626_400000_CN_173582810_400000/LConn1 -- "T_99593626_400000;220000;110000_Stacja_elektroenergetyczna_\"Miłosna\"_400_220_110_kV"/LConn1 -- 400kV_Miłosna___Ołtarzew_CN_99593626_400000_CN_251239544_400000/LConn1 -- 400kV_Miłosna___Stanisławów_CN_99593626_400000_CN_255972397_400000/LConn1 -- 400kV_Miłosna___Stanisławów_CN_99593626_400000_CN_255973806_400000/LConn1 -- 400kV_Miłosna___Ołtarzew_CN_99593626_400000_CN_91384044_400000/LConn1
  400kV_Kozienice___Miłosna_CN_99593626_400000_CN_173582810_400000/LConn2 -- "T_99593626_400000;220000;110000_Stacja_elektroenergetyczna_\"Miłosna\"_400_220_110_kV"/LConn2 -- 400kV_Miłosna___Ołtarzew_CN_99593626_400000_CN_251239544_400000/LConn2 -- 400kV_Miłosna___Stanisławów_CN_99593626_400000_CN_255972397_400000/LConn2 -- 400kV_Miłosna___Stanisławów_CN_99593626_400000_CN_255973806_400000/LConn2 -- 400kV_Miłosna___Ołtarzew_CN_99593626_400000_CN_91384044_400000/LConn2
  400kV_Kozienice___Miłosna_CN_99593626_400000_CN_173582810_400000/LConn3 -- "T_99593626_400000;220000;110000_Stacja_elektroenergetyczna_\"Miłosna\"_400_220_110_kV"/LConn3 -- 400kV_Miłosna___Ołtarzew_CN_99593626_400000_CN_251239544_400000/LConn3 -- bus134/LConn1 -- 400kV_Miłosna___Stanisławów_CN_99593626_400000_CN_255972397_400000/LConn3 -- 400kV_Miłosna___Stanisławów_CN_99593626_400000_CN_255973806_400000/LConn3 -- 400kV_Miłosna___Ołtarzew_CN_99593626_400000_CN_91384044_400000/LConn3
  400kV_Kozienice___Miłosna_CN_99593626_400000_CN_173582810_400000/RConn1 -- "T_173582810_400000;220000;110000_Stacja_elektroenergetyczna_\"Kozienice\"_400_220_110_kV"/LConn1 -- 400kV_Kozienice___Lublin_CN_148060965_400000_CN_173582810_400000/LConn1
  400kV_Kozienice___Miłosna_CN_99593626_400000_CN_173582810_400000/RConn2 -- "T_173582810_400000;220000;110000_Stacja_elektroenergetyczna_\"Kozienice\"_400_220_110_kV"/LConn2 -- 400kV_Kozienice___Lublin_CN_148060965_400000_CN_173582810_400000/LConn2
  400kV_Kozienice___Miłosna_CN_99593626_400000_CN_173582810_400000/RConn3 -- "T_173582810_400000;220000;110000_Stacja_elektroenergetyczna_\"Kozienice\"_400_220_110_kV"/LConn3 -- 400kV_Kozienice___Lublin_CN_148060965_400000_CN_173582810_400000/LConn3 -- bus135/LConn1
  "T_255972397_400000;110000_Stacja_elektroenergetyczna_400_110kV_\"Siedlce_Ujrzanów\""/LConn1 -- 400kV_Miłosna___Stanisławów_CN_99593626_400000_CN_255972397_400000/RConn1
  "T_255972397_400000;110000_Stacja_elektroenergetyczna_400_110kV_\"Siedlce_Ujrzanów\""/LConn2 -- 400kV_Miłosna___Stanisławów_CN_99593626_400000_CN_255972397_400000/RConn2
  400kV_Miłosna___Stanisławów_CN_99593626_400000_CN_255972397_400000/RConn3 -- "T_255972397_400000;110000_Stacja_elektroenergetyczna_400_110kV_\"Siedlce_Ujrzanów\""/LConn3 -- bus136/LConn1
  400kV_Miłosna___Stanisławów_CN_99593626_400000_CN_255973806_400000/RConn1 -- "T_255973806_400000_Stacja_elektrenergetyczna_400kV_\"Stanisławów\""/LConn1 -- 400kV_Miłosna___Narew_CN_255973806_400000_CN_293489663_400000/LConn1 -- 400kV_Miłosna___Narew_CN_255973806_400000_CN_255972326_400000/LConn1
  400kV_Miłosna___Stanisławów_CN_99593626_400000_CN_255973806_400000/RConn2 -- "T_255973806_400000_Stacja_elektrenergetyczna_400kV_\"Stanisławów\""/LConn2 -- 400kV_Miłosna___Narew_CN_255973806_400000_CN_293489663_400000/LConn2 -- 400kV_Miłosna___Narew_CN_255973806_400000_CN_255972326_400000/LConn2
  400kV_Miłosna___Stanisławów_CN_99593626_400000_CN_255973806_400000/RConn3 -- "T_255973806_400000_Stacja_elektrenergetyczna_400kV_\"Stanisławów\""/LConn3 -- 400kV_Miłosna___Narew_CN_255973806_400000_CN_293489663_400000/LConn3 -- bus137/LConn1 -- 400kV_Miłosna___Narew_CN_255973806_400000_CN_255972326_400000/LConn3
  "T_91384044_400000;110000_Stacja_elektroenergetyczna_\"Mościska\"_400_110_kV"/LConn1 -- 400kV_Miłosna___Ołtarzew_CN_99593626_400000_CN_91384044_400000/RConn1
  "T_91384044_400000;110000_Stacja_elektroenergetyczna_\"Mościska\"_400_110_kV"/LConn2 -- 400kV_Miłosna___Ołtarzew_CN_99593626_400000_CN_91384044_400000/RConn2
  400kV_Miłosna___Ołtarzew_CN_99593626_400000_CN_91384044_400000/RConn3 -- "T_91384044_400000;110000_Stacja_elektroenergetyczna_\"Mościska\"_400_110_kV"/LConn3 -- bus138/LConn1
  400kV_Miłosna___Ołtarzew_CN_99593626_400000_CN_251239544_400000/RConn1 -- "T_251239544_400000;220000;110000_Stacja_elektroenergetyczna_\"Ołtarzew\"_400_220_110kV"/LConn1 -- 400kV_Rogowiec___Płock_CN_144646702_400000_CN_251239544_400000/RConn1
  400kV_Miłosna___Ołtarzew_CN_99593626_400000_CN_251239544_400000/RConn2 -- "T_251239544_400000;220000;110000_Stacja_elektroenergetyczna_\"Ołtarzew\"_400_220_110kV"/LConn2 -- 400kV_Rogowiec___Płock_CN_144646702_400000_CN_251239544_400000/RConn2
  400kV_Miłosna___Ołtarzew_CN_99593626_400000_CN_251239544_400000/RConn3 -- "T_251239544_400000;220000;110000_Stacja_elektroenergetyczna_\"Ołtarzew\"_400_220_110kV"/LConn3 -- 400kV_Rogowiec___Płock_CN_144646702_400000_CN_251239544_400000/RConn3 -- bus139/LConn1
  T_101914781_400000;220000;110000_Stacja_elektroenergetyczna_„Olsztyn_Mątki”_400_220_110_kV/LConn1 -- 400kV_Gdańsk_Błonia___Olsztyn_Mątki_CN_101914781_400000_CN_112614319_400000/RConn1
  T_101914781_400000;220000;110000_Stacja_elektroenergetyczna_„Olsztyn_Mątki”_400_220_110_kV/LConn2 -- 400kV_Gdańsk_Błonia___Olsztyn_Mątki_CN_101914781_400000_CN_112614319_400000/RConn2
  400kV_Gdańsk_Błonia___Olsztyn_Mątki_CN_101914781_400000_CN_112614319_400000/RConn3 -- T_101914781_400000;220000;110000_Stacja_elektroenergetyczna_„Olsztyn_Mątki”_400_220_110_kV/LConn3 -- bus140/LConn1
  "T_276291999__Stacja_elektroenergetyczna_\"Świebodzice\"_400_kV"/LConn1 -- Świebodzice___Wrocław_CN_276291999_400000_CN_154510504_400000/RConn1
  "T_276291999__Stacja_elektroenergetyczna_\"Świebodzice\"_400_kV"/LConn2 -- Świebodzice___Wrocław_CN_276291999_400000_CN_154510504_400000/RConn2
  Świebodzice___Wrocław_CN_276291999_400000_CN_154510504_400000/RConn3 -- "T_276291999__Stacja_elektroenergetyczna_\"Świebodzice\"_400_kV"/LConn3 -- bus141/LConn1
  400kV_Kozienice___Lublin_CN_148060965_400000_CN_254235846_400000/LConn1 -- "T_148060965_400000;110000_Stacja_elektroenergetyczna_\"Lublin\"_400_110kV"/LConn1 -- 400kV_Kozienice___Lublin_CN_148060965_400000_CN_173582810_400000/RConn1
  400kV_Kozienice___Lublin_CN_148060965_400000_CN_254235846_400000/LConn2 -- "T_148060965_400000;110000_Stacja_elektroenergetyczna_\"Lublin\"_400_110kV"/LConn2 -- 400kV_Kozienice___Lublin_CN_148060965_400000_CN_173582810_400000/RConn2
  400kV_Kozienice___Lublin_CN_148060965_400000_CN_254235846_400000/LConn3 -- "T_148060965_400000;110000_Stacja_elektroenergetyczna_\"Lublin\"_400_110kV"/LConn3 -- 400kV_Kozienice___Lublin_CN_148060965_400000_CN_173582810_400000/RConn3 -- bus142/LConn1
  400kV_Kozienice___Lublin_CN_148060965_400000_CN_254235846_400000/RConn1 -- "T_254235846_400000;110000_Stacja_elektroenergetyczna_\"Ostrowiec\"_400_110_kV"/LConn1 -- 400_kV_Połaniec_Ostrowiec_CN_199098053_400000_CN_254235846_400000/LConn1
  400kV_Kozienice___Lublin_CN_148060965_400000_CN_254235846_400000/RConn2 -- "T_254235846_400000;110000_Stacja_elektroenergetyczna_\"Ostrowiec\"_400_110_kV"/LConn2 -- 400_kV_Połaniec_Ostrowiec_CN_199098053_400000_CN_254235846_400000/LConn2
  400kV_Kozienice___Lublin_CN_148060965_400000_CN_254235846_400000/RConn3 -- "T_254235846_400000;110000_Stacja_elektroenergetyczna_\"Ostrowiec\"_400_110_kV"/LConn3 -- 400_kV_Połaniec_Ostrowiec_CN_199098053_400000_CN_254235846_400000/LConn3 -- bus143/LConn1
  "T_303870256_400000_Stacja_elektroenergetyczna_\"Ełk_Bis\"_400_kV"/LConn1 -- 400kV_Ełk___Łomża_CN_303870256_400000_CN_255972326_400000/LConn1
  "T_303870256_400000_Stacja_elektroenergetyczna_\"Ełk_Bis\"_400_kV"/LConn2 -- 400kV_Ełk___Łomża_CN_303870256_400000_CN_255972326_400000/LConn2
  400kV_Ełk___Łomża_CN_303870256_400000_CN_255972326_400000/LConn3 -- "T_303870256_400000_Stacja_elektroenergetyczna_\"Ełk_Bis\"_400_kV"/LConn3 -- bus144/LConn1
  400kV_Ełk___Łomża_CN_303870256_400000_CN_255972326_400000/RConn1 -- "T_255972326_400000_Stacja_elektrenergetyczna_400kV_\"Łomża\""/LConn1 -- 400kV_Miłosna___Narew_CN_255973806_400000_CN_255972326_400000/RConn1 -- 400kV_Ostrołęka___Łomża_CN_255972326_400000_CN_121656686_400000/LConn1
  400kV_Ełk___Łomża_CN_303870256_400000_CN_255972326_400000/RConn2 -- "T_255972326_400000_Stacja_elektrenergetyczna_400kV_\"Łomża\""/LConn2 -- 400kV_Miłosna___Narew_CN_255973806_400000_CN_255972326_400000/RConn2 -- 400kV_Ostrołęka___Łomża_CN_255972326_400000_CN_121656686_400000/LConn2
  400kV_Ełk___Łomża_CN_303870256_400000_CN_255972326_400000/RConn3 -- "T_255972326_400000_Stacja_elektrenergetyczna_400kV_\"Łomża\""/LConn3 -- 400kV_Miłosna___Narew_CN_255973806_400000_CN_255972326_400000/RConn3 -- 400kV_Ostrołęka___Łomża_CN_255972326_400000_CN_121656686_400000/LConn3 -- bus145/LConn1
  T_293489663_400000;110000_Stacja_elektroenergetyczna_„Narew”_400_110_kV/LConn1 -- 400kV_Miłosna___Narew_CN_255973806_400000_CN_293489663_400000/RConn1
  T_293489663_400000;110000_Stacja_elektroenergetyczna_„Narew”_400_110_kV/LConn2 -- 400kV_Miłosna___Narew_CN_255973806_400000_CN_293489663_400000/RConn2
  400kV_Miłosna___Narew_CN_255973806_400000_CN_293489663_400000/RConn3 -- T_293489663_400000;110000_Stacja_elektroenergetyczna_„Narew”_400_110_kV/LConn3 -- bus146/LConn1
  "T_199098050_400000;220000_Stacja_elektroenergetyczna_\"Kielce\"_400_220kV"/LConn1 -- 400_kV_Połaniec___Kielce_CN_199098050_400000_CN_199098053_400000/LConn1
  "T_199098050_400000;220000_Stacja_elektroenergetyczna_\"Kielce\"_400_220kV"/LConn2 -- 400_kV_Połaniec___Kielce_CN_199098050_400000_CN_199098053_400000/LConn2
  400_kV_Połaniec___Kielce_CN_199098050_400000_CN_199098053_400000/LConn3 -- "T_199098050_400000;220000_Stacja_elektroenergetyczna_\"Kielce\"_400_220kV"/LConn3 -- bus147/LConn1
  400_kV_Połaniec___Kielce_CN_199098050_400000_CN_199098053_400000/RConn1 -- "T_199098053_400000;220000;110000;15000_Stacja_elektroenergetyczna_\"Połaniec\"_400_220_110kV"/LConn1 -- 400_kV_Tarnów___Krosno_Iskrzynia_CN_166838338_400000_CN_199098053_400000/LConn1 -- _CN_199098053_400000_CN_130207099_220000/RConn1 -- 400_kV_Połaniec_Ostrowiec_CN_199098053_400000_CN_254235846_400000/RConn1
  400_kV_Połaniec___Kielce_CN_199098050_400000_CN_199098053_400000/RConn2 -- "T_199098053_400000;220000;110000;15000_Stacja_elektroenergetyczna_\"Połaniec\"_400_220_110kV"/LConn2 -- 400_kV_Tarnów___Krosno_Iskrzynia_CN_166838338_400000_CN_199098053_400000/LConn2 -- _CN_199098053_400000_CN_130207099_220000/RConn2 -- 400_kV_Połaniec_Ostrowiec_CN_199098053_400000_CN_254235846_400000/RConn2
  400_kV_Połaniec___Kielce_CN_199098050_400000_CN_199098053_400000/RConn3 -- "T_199098053_400000;220000;110000;15000_Stacja_elektroenergetyczna_\"Połaniec\"_400_220_110kV"/LConn3 -- 400_kV_Tarnów___Krosno_Iskrzynia_CN_166838338_400000_CN_199098053_400000/LConn3 -- _CN_199098053_400000_CN_130207099_220000/RConn3 -- 400_kV_Połaniec_Ostrowiec_CN_199098053_400000_CN_254235846_400000/RConn3 -- bus148/LConn1
  400_kV_Tarnów___Krosno_Iskrzynia_CN_166838338_400000_CN_166710856_400000/LConn1 -- "T_166838338_400000;110000_Stacja_elektroenergetyczna_\"Krosno_Iskrzynia\"_400_110_kV"/LConn1 -- 400_kV_Tarnów___Krosno_Iskrzynia_CN_166838338_400000_CN_40946784_400000/RConn1 -- 400_kV_Tarnów___Krosno_Iskrzynia_CN_166838338_400000_CN_199098053_400000/RConn1 -- 400_kV_Tarnów___Krosno_Iskrzynia_CN_166838338_400000_CN_215282393_400000/LConn1
  400_kV_Tarnów___Krosno_Iskrzynia_CN_166838338_400000_CN_166710856_400000/LConn2 -- "T_166838338_400000;110000_Stacja_elektroenergetyczna_\"Krosno_Iskrzynia\"_400_110_kV"/LConn2 -- 400_kV_Tarnów___Krosno_Iskrzynia_CN_166838338_400000_CN_40946784_400000/RConn2 -- 400_kV_Tarnów___Krosno_Iskrzynia_CN_166838338_400000_CN_199098053_400000/RConn2 -- 400_kV_Tarnów___Krosno_Iskrzynia_CN_166838338_400000_CN_215282393_400000/LConn2
  400_kV_Tarnów___Krosno_Iskrzynia_CN_166838338_400000_CN_166710856_400000/LConn3 -- "T_166838338_400000;110000_Stacja_elektroenergetyczna_\"Krosno_Iskrzynia\"_400_110_kV"/LConn3 -- 400_kV_Tarnów___Krosno_Iskrzynia_CN_166838338_400000_CN_40946784_400000/RConn3 -- 400_kV_Tarnów___Krosno_Iskrzynia_CN_166838338_400000_CN_199098053_400000/RConn3 -- 400_kV_Tarnów___Krosno_Iskrzynia_CN_166838338_400000_CN_215282393_400000/LConn3 -- bus149/LConn1
  T_166710856_400000;110000_Stacja_elektroenergetyczna_„Tarnów”_400_110_kV/LConn1 -- 400_kV_Tarnów___Krosno_Iskrzynia_CN_166838338_400000_CN_166710856_400000/RConn1
  T_166710856_400000;110000_Stacja_elektroenergetyczna_„Tarnów”_400_110_kV/LConn2 -- 400_kV_Tarnów___Krosno_Iskrzynia_CN_166838338_400000_CN_166710856_400000/RConn2
  400_kV_Tarnów___Krosno_Iskrzynia_CN_166838338_400000_CN_166710856_400000/RConn3 -- T_166710856_400000;110000_Stacja_elektroenergetyczna_„Tarnów”_400_110_kV/LConn3 -- bus150/LConn1
  T_215282393_750000;400000;110000_Rzeszów_Systemowa_(Widełka)_750_400_110_kV/LConn1 -- 400_kV_Tarnów___Krosno_Iskrzynia_CN_166838338_400000_CN_215282393_400000/RConn1
  T_215282393_750000;400000;110000_Rzeszów_Systemowa_(Widełka)_750_400_110_kV/LConn2 -- 400_kV_Tarnów___Krosno_Iskrzynia_CN_166838338_400000_CN_215282393_400000/RConn2
  400_kV_Tarnów___Krosno_Iskrzynia_CN_166838338_400000_CN_215282393_400000/RConn3 -- T_215282393_750000;400000;110000_Rzeszów_Systemowa_(Widełka)_750_400_110_kV/LConn3 -- bus151/LConn1
  "T_121656686_400000;220000;110000_Stacja_elektroenergetyczna_400_220_110kV_\"Ostrołęka\""/LConn1 -- 400kV_Ostrołęka___Łomża_CN_255972326_400000_CN_121656686_400000/RConn1
  "T_121656686_400000;220000;110000_Stacja_elektroenergetyczna_400_220_110kV_\"Ostrołęka\""/LConn2 -- 400kV_Ostrołęka___Łomża_CN_255972326_400000_CN_121656686_400000/RConn2
  400kV_Ostrołęka___Łomża_CN_255972326_400000_CN_121656686_400000/RConn3 -- "T_121656686_400000;220000;110000_Stacja_elektroenergetyczna_400_220_110kV_\"Ostrołęka\""/LConn3 -- bus152/LConn1
  400kV_Mikułowa___Czarna_CN_154894455_400000_CN_111615226_400000/RConn1 -- T_111615226_400000;220000;110000_Stacja_elektroenergetyczna_„Mikułowa”_400_220_110_kV/LConn1 -- 400kV_Turów___Mikułowa_CN_111615226_400000_CN_90038401_220000/RConn1
  400kV_Mikułowa___Czarna_CN_154894455_400000_CN_111615226_400000/RConn2 -- T_111615226_400000;220000;110000_Stacja_elektroenergetyczna_„Mikułowa”_400_220_110_kV/LConn2 -- 400kV_Turów___Mikułowa_CN_111615226_400000_CN_90038401_220000/RConn2
  400kV_Mikułowa___Czarna_CN_154894455_400000_CN_111615226_400000/RConn3 -- T_111615226_400000;220000;110000_Stacja_elektroenergetyczna_„Mikułowa”_400_220_110_kV/LConn3 -- 400kV_Turów___Mikułowa_CN_111615226_400000_CN_90038401_220000/RConn3 -- bus153/LConn1
  "T_87667718_220000;110000_Stacja_elektroenergetyczna_\"Lubocza\"_220_110kV"/RConn1 -- L_87667718/LConn1
  "T_87667718_220000;110000_Stacja_elektroenergetyczna_\"Lubocza\"_220_110kV"/RConn2 -- L_87667718/LConn2
  L_87667718/LConn3 -- "T_87667718_220000;110000_Stacja_elektroenergetyczna_\"Lubocza\"_220_110kV"/RConn3 -- bus154/LConn1
  "T_191035265_220000;110000_Stacja_elektroenergetyczna_\"Klikowa\"_220_110_kV"/RConn1 -- L_191035265/LConn1
  "T_191035265_220000;110000_Stacja_elektroenergetyczna_\"Klikowa\"_220_110_kV"/RConn2 -- L_191035265/LConn2
  L_191035265/LConn3 -- "T_191035265_220000;110000_Stacja_elektroenergetyczna_\"Klikowa\"_220_110_kV"/RConn3 -- bus155/LConn1
  T_115801644_220000;110000_Stacja_elektroenergetyczna_„Wanda”_220_110_kV/RConn1 -- L_115801644/LConn1
  T_115801644_220000;110000_Stacja_elektroenergetyczna_„Wanda”_220_110_kV/RConn2 -- L_115801644/LConn2
  L_115801644/LConn3 -- T_115801644_220000;110000_Stacja_elektroenergetyczna_„Wanda”_220_110_kV/RConn3 -- bus156/LConn1
  T_187420591_220000;110000_Stacja_elektroenergetyczna_„Siersza”_220_110kV/RConn1 -- L_187420591/LConn1
  T_187420591_220000;110000_Stacja_elektroenergetyczna_„Siersza”_220_110kV/RConn2 -- L_187420591/LConn2
  L_187420591/LConn3 -- T_187420591_220000;110000_Stacja_elektroenergetyczna_„Siersza”_220_110kV/RConn3 -- bus157/LConn1
  "T_223873553_220000;110000_Stacja_elektroenergetyczna_\"Gorzów\"_220_110_kV"/RConn1 -- L_223873553/LConn1
  "T_223873553_220000;110000_Stacja_elektroenergetyczna_\"Gorzów\"_220_110_kV"/RConn2 -- L_223873553/LConn2
  L_223873553/LConn3 -- "T_223873553_220000;110000_Stacja_elektroenergetyczna_\"Gorzów\"_220_110_kV"/RConn3 -- bus158/LConn1
  "T_158232924_220000;110000_Stacja_elektroenergetyczna_\"Leśniów\"_220_110_kV"/RConn1 -- L_158232924/LConn1
  "T_158232924_220000;110000_Stacja_elektroenergetyczna_\"Leśniów\"_220_110_kV"/RConn2 -- L_158232924/LConn2
  L_158232924/LConn3 -- "T_158232924_220000;110000_Stacja_elektroenergetyczna_\"Leśniów\"_220_110_kV"/RConn3 -- bus159/LConn1
  T_171383831_220000;110000_Stacja_elektroenergetyczna_Adamów_220_110_kV/RConn1 -- L_171383831/LConn1
  T_171383831_220000;110000_Stacja_elektroenergetyczna_Adamów_220_110_kV/RConn2 -- L_171383831/LConn2
  L_171383831/LConn3 -- T_171383831_220000;110000_Stacja_elektroenergetyczna_Adamów_220_110_kV/RConn3 -- bus160/LConn1
  "T_216975352_220000;110000_Stacja_elektroenergetyczna_\"Konin\"_220_110_kV"/RConn1 -- L_216975352/LConn1
  "T_216975352_220000;110000_Stacja_elektroenergetyczna_\"Konin\"_220_110_kV"/RConn2 -- L_216975352/LConn2
  L_216975352/LConn3 -- "T_216975352_220000;110000_Stacja_elektroenergetyczna_\"Konin\"_220_110_kV"/RConn3 -- bus161/LConn1
  "T_35366436_220000;110000_Stacja_elektroenergetyczna_\"Janów\"_220_110_kV"/RConn1 -- L_35366436/LConn1
  "T_35366436_220000;110000_Stacja_elektroenergetyczna_\"Janów\"_220_110_kV"/RConn2 -- L_35366436/LConn2
  L_35366436/LConn3 -- "T_35366436_220000;110000_Stacja_elektroenergetyczna_\"Janów\"_220_110_kV"/RConn3 -- bus162/LConn1
  T_101982559_220000;110000_Stacja_elektroenergetyczna_„Zgierz”_220_110_kV/RConn1 -- L_101982559/LConn1
  T_101982559_220000;110000_Stacja_elektroenergetyczna_„Zgierz”_220_110_kV/RConn2 -- L_101982559/LConn2
  L_101982559/LConn3 -- T_101982559_220000;110000_Stacja_elektroenergetyczna_„Zgierz”_220_110_kV/RConn3 -- bus163/LConn1
  "T_102165724_220000;110000_Stacja_elektroenergetyczna_\"Pabianice\"_220_110_kV"/RConn1 -- L_102165724/LConn1
  "T_102165724_220000;110000_Stacja_elektroenergetyczna_\"Pabianice\"_220_110_kV"/RConn2 -- L_102165724/LConn2
  L_102165724/LConn3 -- "T_102165724_220000;110000_Stacja_elektroenergetyczna_\"Pabianice\"_220_110_kV"/RConn3 -- bus164/LConn1
  T_385098015__Stacja_elektroenergetyczna_400_110_kV_Pelplin/RConn1 -- L_385098015/LConn1
  T_385098015__Stacja_elektroenergetyczna_400_110_kV_Pelplin/RConn2 -- L_385098015/LConn2
  L_385098015/LConn3 -- T_385098015__Stacja_elektroenergetyczna_400_110_kV_Pelplin/RConn3 -- bus165/LConn1
  "T_178838661_220000;110000_Stacja_elektroenergetyczna_\"Żydowo\"_220_110_kV"/RConn1 -- L_178838661/LConn1
  "T_178838661_220000;110000_Stacja_elektroenergetyczna_\"Żydowo\"_220_110_kV"/RConn2 -- L_178838661/LConn2
  L_178838661/LConn3 -- "T_178838661_220000;110000_Stacja_elektroenergetyczna_\"Żydowo\"_220_110_kV"/RConn3 -- bus166/LConn1
  T_170316833_220000;110000_Stacja_elektroenergetyczna_„Piotrków”_220_110_kV/RConn1 -- L_170316833/LConn1
  T_170316833_220000;110000_Stacja_elektroenergetyczna_„Piotrków”_220_110_kV/RConn2 -- L_170316833/LConn2
  L_170316833/LConn3 -- T_170316833_220000;110000_Stacja_elektroenergetyczna_„Piotrków”_220_110_kV/RConn3 -- bus167/LConn1
  "T_255284259_220000;110000_Stacja_elektroenergetyczna_\"Pątnów\"_220_110_kV"/RConn1 -- L_255284259/LConn1
  "T_255284259_220000;110000_Stacja_elektroenergetyczna_\"Pątnów\"_220_110_kV"/RConn2 -- L_255284259/LConn2
  L_255284259/LConn3 -- "T_255284259_220000;110000_Stacja_elektroenergetyczna_\"Pątnów\"_220_110_kV"/RConn3 -- bus168/LConn1
  "T_180824706_220000;110000_Stacja_elektroenergetyczna_\"Czerwonak\"_220_110_kV"/RConn1 -- L_180824706/LConn1
  "T_180824706_220000;110000_Stacja_elektroenergetyczna_\"Czerwonak\"_220_110_kV"/RConn2 -- L_180824706/LConn2
  L_180824706/LConn3 -- "T_180824706_220000;110000_Stacja_elektroenergetyczna_\"Czerwonak\"_220_110_kV"/RConn3 -- bus169/LConn1
  "T_29115701_220000;110000_Stacja_elektroenergetyczna_\"Mory\"_220_110kV"/RConn1 -- L_29115701/LConn1
  "T_29115701_220000;110000_Stacja_elektroenergetyczna_\"Mory\"_220_110kV"/RConn2 -- L_29115701/LConn2
  L_29115701/LConn3 -- "T_29115701_220000;110000_Stacja_elektroenergetyczna_\"Mory\"_220_110kV"/RConn3 -- bus170/LConn1
  "T_171992870_220000;110000_Stacja_elektroenergetyczna_\"Podolszyce\"_220_110kV"/RConn1 -- L_171992870/LConn1
  "T_171992870_220000;110000_Stacja_elektroenergetyczna_\"Podolszyce\"_220_110kV"/RConn2 -- L_171992870/LConn2
  L_171992870/LConn3 -- "T_171992870_220000;110000_Stacja_elektroenergetyczna_\"Podolszyce\"_220_110kV"/RConn3 -- bus171/LConn1
  "T_72879943_220000;110000_Stacja_elektroenergetyczna_\"Włocławek_Azoty\"_220_110_kV"/RConn1 -- L_72879943/LConn1
  "T_72879943_220000;110000_Stacja_elektroenergetyczna_\"Włocławek_Azoty\"_220_110_kV"/RConn2 -- L_72879943/LConn2
  L_72879943/LConn3 -- "T_72879943_220000;110000_Stacja_elektroenergetyczna_\"Włocławek_Azoty\"_220_110_kV"/RConn3 -- bus172/LConn1
  "T_46235456_220000;110000_Stacja_elektroenergetyczna_\"Jasiniec\"_220_110_kV"/RConn1 -- L_46235456/LConn1
  "T_46235456_220000;110000_Stacja_elektroenergetyczna_\"Jasiniec\"_220_110_kV"/RConn2 -- L_46235456/LConn2
  L_46235456/LConn3 -- "T_46235456_220000;110000_Stacja_elektroenergetyczna_\"Jasiniec\"_220_110_kV"/RConn3 -- bus173/LConn1
  "T_44389929_220000_Stacja_elektroenergetyczna_\"Bujaków\"_220kV"/RConn1 -- L_44389929/LConn1
  "T_44389929_220000_Stacja_elektroenergetyczna_\"Bujaków\"_220kV"/RConn2 -- L_44389929/LConn2
  L_44389929/LConn3 -- "T_44389929_220000_Stacja_elektroenergetyczna_\"Bujaków\"_220kV"/RConn3 -- bus174/LConn1
  "T_98634956_220000;110000_Stacja_elektroenergetyczna_\"Komorowice\"_220_110_kV"/RConn1 -- L_98634956/LConn1
  "T_98634956_220000;110000_Stacja_elektroenergetyczna_\"Komorowice\"_220_110_kV"/RConn2 -- L_98634956/LConn2
  L_98634956/LConn3 -- "T_98634956_220000;110000_Stacja_elektroenergetyczna_\"Komorowice\"_220_110_kV"/RConn3 -- bus175/LConn1
  T_291375946__Stacja_elektroenergetyczna_„Czeczot”_220_110_kV/RConn1 -- L_291375946/LConn1
  T_291375946__Stacja_elektroenergetyczna_„Czeczot”_220_110_kV/RConn2 -- L_291375946/LConn2
  L_291375946/LConn3 -- T_291375946__Stacja_elektroenergetyczna_„Czeczot”_220_110_kV/RConn3 -- bus176/LConn1
  T_135598292_220000;110000_Stacja_elektroenergetyczna_„Poręba”_220_110_kV/RConn1 -- L_135598292/LConn1
  T_135598292_220000;110000_Stacja_elektroenergetyczna_„Poręba”_220_110_kV/RConn2 -- L_135598292/LConn2
  L_135598292/LConn3 -- T_135598292_220000;110000_Stacja_elektroenergetyczna_„Poręba”_220_110_kV/RConn3 -- bus177/LConn1
  "T_255232597_220000;110000_Stacja_elektroenergetyczna_\"Bieruń\"_220_110_kV"/RConn1 -- L_255232597/LConn1
  "T_255232597_220000;110000_Stacja_elektroenergetyczna_\"Bieruń\"_220_110_kV"/RConn2 -- L_255232597/LConn2
  L_255232597/LConn3 -- "T_255232597_220000;110000_Stacja_elektroenergetyczna_\"Bieruń\"_220_110_kV"/RConn3 -- bus178/LConn1
  T_133537926_220000_Stacja_elektroenergetyczna_„Byczyna”_220_kV/RConn1 -- L_133537926/LConn1
  T_133537926_220000_Stacja_elektroenergetyczna_„Byczyna”_220_kV/RConn2 -- L_133537926/LConn2
  L_133537926/LConn3 -- T_133537926_220000_Stacja_elektroenergetyczna_„Byczyna”_220_kV/RConn3 -- bus179/LConn1
  T_184899160_220000;110000_Stacja_elektroenergetyczna_„Moszczenica”_220_110_kV/RConn1 -- L_184899160/LConn1
  T_184899160_220000;110000_Stacja_elektroenergetyczna_„Moszczenica”_220_110_kV/RConn2 -- L_184899160/LConn2
  L_184899160/LConn3 -- T_184899160_220000;110000_Stacja_elektroenergetyczna_„Moszczenica”_220_110_kV/RConn3 -- bus180/LConn1
  "T_183945016_220000;110000_Stacja_elektroenergetyczna_\"Kopanina\"_220_110_kV"/RConn1 -- L_183945016/LConn1
  "T_183945016_220000;110000_Stacja_elektroenergetyczna_\"Kopanina\"_220_110_kV"/RConn2 -- L_183945016/LConn2
  L_183945016/LConn3 -- "T_183945016_220000;110000_Stacja_elektroenergetyczna_\"Kopanina\"_220_110_kV"/RConn3 -- bus181/LConn1
  "T_135175732__Stacja_elektroenergetyczna_\"Biskupice\"_220_110kV"/RConn1 -- L_135175732/LConn1
  "T_135175732__Stacja_elektroenergetyczna_\"Biskupice\"_220_110kV"/RConn2 -- L_135175732/LConn2
  L_135175732/LConn3 -- "T_135175732__Stacja_elektroenergetyczna_\"Biskupice\"_220_110kV"/RConn3 -- bus182/LConn1
  T_179138441_220000;110000_Stacja_elektroenergetyczna_„Świebodzice”_220_110_kV/RConn1 -- L_179138441/LConn1
  T_179138441_220000;110000_Stacja_elektroenergetyczna_„Świebodzice”_220_110_kV/RConn2 -- L_179138441/LConn2
  L_179138441/LConn3 -- T_179138441_220000;110000_Stacja_elektroenergetyczna_„Świebodzice”_220_110_kV/RConn3 -- bus183/LConn1
  "T_180535363_220000;110000_Stacja_elektroenergetyczna_\"Żukowice\"_220_110_kV"/RConn1 -- L_180535363/LConn1
  "T_180535363_220000;110000_Stacja_elektroenergetyczna_\"Żukowice\"_220_110_kV"/RConn2 -- L_180535363/LConn2
  L_180535363/LConn3 -- "T_180535363_220000;110000_Stacja_elektroenergetyczna_\"Żukowice\"_220_110_kV"/RConn3 -- bus184/LConn1
  "T_180542657_220000;110000_Stacja_elektroenergetyczna_\"Polkowice\"_220_110_kV"/RConn1 -- L_180542657/LConn1
  "T_180542657_220000;110000_Stacja_elektroenergetyczna_\"Polkowice\"_220_110_kV"/RConn2 -- L_180542657/LConn2
  L_180542657/LConn3 -- "T_180542657_220000;110000_Stacja_elektroenergetyczna_\"Polkowice\"_220_110_kV"/RConn3 -- bus185/LConn1
  "T_165763717__Stacja_elektroenergetyczna_\"Police\"_220_110kV"/RConn1 -- L_165763717/LConn1
  "T_165763717__Stacja_elektroenergetyczna_\"Police\"_220_110kV"/RConn2 -- L_165763717/LConn2
  L_165763717/LConn3 -- "T_165763717__Stacja_elektroenergetyczna_\"Police\"_220_110kV"/RConn3 -- bus186/LConn1
  T_131120723_220000;110000_Stacja_elektroenergetyczna_220_110_kV_Poznań_Południe/RConn1 -- L_131120723/LConn1
  T_131120723_220000;110000_Stacja_elektroenergetyczna_220_110_kV_Poznań_Południe/RConn2 -- L_131120723/LConn2
  L_131120723/LConn3 -- T_131120723_220000;110000_Stacja_elektroenergetyczna_220_110_kV_Poznań_Południe/RConn3 -- bus187/LConn1
  "T_155971668_220000;110000_Stacja_elektroenergetyczna_\"Kopalnia_Bełchatów\"_220_110kV"/RConn1 -- L_155971668/LConn1
  "T_155971668_220000;110000_Stacja_elektroenergetyczna_\"Kopalnia_Bełchatów\"_220_110kV"/RConn2 -- L_155971668/LConn2
  L_155971668/LConn3 -- "T_155971668_220000;110000_Stacja_elektroenergetyczna_\"Kopalnia_Bełchatów\"_220_110kV"/RConn3 -- bus188/LConn1
  T_173613665_220000;110000_Stacja_elektroenergetyczna_„Zamość”_220_110_kV/RConn1 -- L_173613665/LConn1
  T_173613665_220000;110000_Stacja_elektroenergetyczna_„Zamość”_220_110_kV/RConn2 -- L_173613665/LConn2
  L_173613665/LConn3 -- T_173613665_220000;110000_Stacja_elektroenergetyczna_„Zamość”_220_110_kV/RConn3 -- bus189/LConn1
  T_170368942_220000;110000_Stacja_elektroenergetyczna_„Mokre”_220_110_kV/RConn1 -- L_170368942/LConn1
  T_170368942_220000;110000_Stacja_elektroenergetyczna_„Mokre”_220_110_kV/RConn2 -- L_170368942/LConn2
  L_170368942/LConn3 -- T_170368942_220000;110000_Stacja_elektroenergetyczna_„Mokre”_220_110_kV/RConn3 -- bus190/LConn1
  "T_40946790_220000;110000_Stacja_elektroenergetyczna_\"Jamki\"_220_110kV"/RConn1 -- L_40946790/LConn1
  "T_40946790_220000;110000_Stacja_elektroenergetyczna_\"Jamki\"_220_110kV"/RConn2 -- L_40946790/LConn2
  L_40946790/LConn3 -- "T_40946790_220000;110000_Stacja_elektroenergetyczna_\"Jamki\"_220_110kV"/RConn3 -- bus191/LConn1
  "T_66051759__Stacja_elektroenergetyczna_\"Koksochemia\"_220kV"/RConn1 -- L_66051759/LConn1
  "T_66051759__Stacja_elektroenergetyczna_\"Koksochemia\"_220kV"/RConn2 -- L_66051759/LConn2
  L_66051759/LConn3 -- "T_66051759__Stacja_elektroenergetyczna_\"Koksochemia\"_220kV"/RConn3 -- bus192/LConn1
  "T_191038569__Stacja_elektroenergetyczna_\"Azoty_Tarnów\"_220_110kV"/RConn1 -- L_191038569/LConn1
  "T_191038569__Stacja_elektroenergetyczna_\"Azoty_Tarnów\"_220_110kV"/RConn2 -- L_191038569/LConn2
  L_191038569/LConn3 -- "T_191038569__Stacja_elektroenergetyczna_\"Azoty_Tarnów\"_220_110kV"/RConn3 -- bus193/LConn1
  "T_89434732__Stacja_elektroenergetyczna_\"Towarowa\"_220_110_15kV"/RConn1 -- L_89434732/LConn1
  "T_89434732__Stacja_elektroenergetyczna_\"Towarowa\"_220_110_15kV"/RConn2 -- L_89434732/LConn2
  L_89434732/LConn3 -- "T_89434732__Stacja_elektroenergetyczna_\"Towarowa\"_220_110_15kV"/RConn3 -- bus194/LConn1
  "T_185454704__Stacja_elektroenergetyczna_\"Blachownia\"_220_110kV"/RConn1 -- L_185454704/LConn1
  "T_185454704__Stacja_elektroenergetyczna_\"Blachownia\"_220_110kV"/RConn2 -- L_185454704/LConn2
  L_185454704/LConn3 -- "T_185454704__Stacja_elektroenergetyczna_\"Blachownia\"_220_110kV"/RConn3 -- bus195/LConn1
  "T_185459155__Stacja_elektroenergetyczna_\"Kędzierzyn\"_220_110kV"/RConn1 -- L_185459155/LConn1
  "T_185459155__Stacja_elektroenergetyczna_\"Kędzierzyn\"_220_110kV"/RConn2 -- L_185459155/LConn2
  L_185459155/LConn3 -- "T_185459155__Stacja_elektroenergetyczna_\"Kędzierzyn\"_220_110kV"/RConn3 -- bus196/LConn1
  "T_336990960_220000;110000_Stacja_Energetyczna_\"Groszowice\"_220_110_kV"/RConn1 -- L_336990960/LConn1
  "T_336990960_220000;110000_Stacja_Energetyczna_\"Groszowice\"_220_110_kV"/RConn2 -- L_336990960/LConn2
  L_336990960/LConn3 -- "T_336990960_220000;110000_Stacja_Energetyczna_\"Groszowice\"_220_110_kV"/RConn3 -- bus197/LConn1
  "T_145037309_220000;110000_Stacja_elektroenergetyczna_\"Sochaczew\"_220_110kV"/RConn1 -- L_145037309/LConn1
  "T_145037309_220000;110000_Stacja_elektroenergetyczna_\"Sochaczew\"_220_110kV"/RConn2 -- L_145037309/LConn2
  L_145037309/LConn3 -- "T_145037309_220000;110000_Stacja_elektroenergetyczna_\"Sochaczew\"_220_110kV"/RConn3 -- bus198/LConn1
  "T_216060722_220000;110000_Stacja_elektroenergetyczna_\"Aniołów\"_220_110_kV"/RConn1 -- L_216060722/LConn1
  "T_216060722_220000;110000_Stacja_elektroenergetyczna_\"Aniołów\"_220_110_kV"/RConn2 -- L_216060722/LConn2
  L_216060722/LConn3 -- "T_216060722_220000;110000_Stacja_elektroenergetyczna_\"Aniołów\"_220_110_kV"/RConn3 -- bus199/LConn1
  "T_148197330_220000;110000_Stacja_elektroenergetyczna_\"Leszno\"_220_110_kV"/RConn1 -- L_148197330/LConn1
  "T_148197330_220000;110000_Stacja_elektroenergetyczna_\"Leszno\"_220_110_kV"/RConn2 -- L_148197330/LConn2
  L_148197330/LConn3 -- "T_148197330_220000;110000_Stacja_elektroenergetyczna_\"Leszno\"_220_110_kV"/RConn3 -- bus200/LConn1
  "T_238640596_220000;110000_Stacja_elektroenergetyczna_\"Piła_Krzewina\"_220_110_kV"/RConn1 -- L_238640596/LConn1
  "T_238640596_220000;110000_Stacja_elektroenergetyczna_\"Piła_Krzewina\"_220_110_kV"/RConn2 -- L_238640596/LConn2
  L_238640596/LConn3 -- "T_238640596_220000;110000_Stacja_elektroenergetyczna_\"Piła_Krzewina\"_220_110_kV"/RConn3 -- bus201/LConn1
  "T_40062974_220000;110000_Stacja_elektroenergetyczna_\"Glinki\"_220_110_kV"/RConn1 -- L_40062974/LConn1
  "T_40062974_220000;110000_Stacja_elektroenergetyczna_\"Glinki\"_220_110_kV"/RConn2 -- L_40062974/LConn2
  L_40062974/LConn3 -- "T_40062974_220000;110000_Stacja_elektroenergetyczna_\"Glinki\"_220_110_kV"/RConn3 -- bus202/LConn1
  "T_183259405__Stacja_elektroenergetyczna_\"Halemba\"_220_110kV"/RConn1 -- L_183259405/LConn1
  "T_183259405__Stacja_elektroenergetyczna_\"Halemba\"_220_110kV"/RConn2 -- L_183259405/LConn2
  L_183259405/LConn3 -- "T_183259405__Stacja_elektroenergetyczna_\"Halemba\"_220_110kV"/RConn3 -- bus203/LConn1
  "T_29139402_220000;110000_Stacja_elektroenergetyczna_\"Katowice\"_220_110_kV"/RConn1 -- L_29139402/LConn1
  "T_29139402_220000;110000_Stacja_elektroenergetyczna_\"Katowice\"_220_110_kV"/RConn2 -- L_29139402/LConn2
  L_29139402/LConn3 -- "T_29139402_220000;110000_Stacja_elektroenergetyczna_\"Katowice\"_220_110_kV"/RConn3 -- bus204/LConn1
  "T_88544449__Stacja_elektroenergetyczna_\"Puławy\"_220kV"/RConn1 -- L_88544449/LConn1
  "T_88544449__Stacja_elektroenergetyczna_\"Puławy\"_220kV"/RConn2 -- L_88544449/LConn2
  L_88544449/LConn3 -- "T_88544449__Stacja_elektroenergetyczna_\"Puławy\"_220kV"/RConn3 -- bus205/LConn1
  "T_170249563_220000;110000_Stacja_elektroenergetyczna_\"Abramowice\"_220_110_kV"/RConn1 -- L_170249563/LConn1
  "T_170249563_220000;110000_Stacja_elektroenergetyczna_\"Abramowice\"_220_110_kV"/RConn2 -- L_170249563/LConn2
  L_170249563/LConn3 -- "T_170249563_220000;110000_Stacja_elektroenergetyczna_\"Abramowice\"_220_110_kV"/RConn3 -- bus206/LConn1
  T_189851841_220000;110000_Stacja_elektroenergetyczna_„Rożki”_220_110_kV/RConn1 -- L_189851841/LConn1
  T_189851841_220000;110000_Stacja_elektroenergetyczna_„Rożki”_220_110_kV/RConn2 -- L_189851841/LConn2
  L_189851841/LConn3 -- T_189851841_220000;110000_Stacja_elektroenergetyczna_„Rożki”_220_110_kV/RConn3 -- bus207/LConn1
  T_143484238_220000;110000_Stacja_elektroenergetyczna_„Toruń___Elana”_220_110_kV/RConn1 -- L_143484238/LConn1
  T_143484238_220000;110000_Stacja_elektroenergetyczna_„Toruń___Elana”_220_110_kV/RConn2 -- L_143484238/LConn2
  L_143484238/LConn3 -- T_143484238_220000;110000_Stacja_elektroenergetyczna_„Toruń___Elana”_220_110_kV/RConn3 -- bus208/LConn1
  T_101915790_220000;110000;15000_Stacja_elektroenergetyczna_„Olsztyn_I”_220_110_15_kV/RConn1 -- L_101915790/LConn1
  T_101915790_220000;110000;15000_Stacja_elektroenergetyczna_„Olsztyn_I”_220_110_15_kV/RConn2 -- L_101915790/LConn2
  L_101915790/LConn3 -- T_101915790_220000;110000;15000_Stacja_elektroenergetyczna_„Olsztyn_I”_220_110_15_kV/RConn3 -- bus209/LConn1
  "T_170259740_220000;110000_Stacja_elektroenergetyczna_\"Ełk\"_220_110_kV"/RConn1 -- L_170259740/LConn1
  "T_170259740_220000;110000_Stacja_elektroenergetyczna_\"Ełk\"_220_110_kV"/RConn2 -- L_170259740/LConn2
  L_170259740/LConn3 -- "T_170259740_220000;110000_Stacja_elektroenergetyczna_\"Ełk\"_220_110_kV"/RConn3 -- bus210/LConn1
  "T_178756295_220000;110000_Stacja_elektroenergetyczna_\"Cieplice\"_220_110_kV"/RConn1 -- L_178756295/LConn1
  "T_178756295_220000;110000_Stacja_elektroenergetyczna_\"Cieplice\"_220_110_kV"/RConn2 -- L_178756295/LConn2
  L_178756295/LConn3 -- "T_178756295_220000;110000_Stacja_elektroenergetyczna_\"Cieplice\"_220_110_kV"/RConn3 -- bus211/LConn1
  "T_177749653_220000;110000_Stacja_elektroenergetyczna_\"Boguszów\"_220_110_kV"/RConn1 -- L_177749653/LConn1
  "T_177749653_220000;110000_Stacja_elektroenergetyczna_\"Boguszów\"_220_110_kV"/RConn2 -- L_177749653/LConn2
  L_177749653/LConn3 -- "T_177749653_220000;110000_Stacja_elektroenergetyczna_\"Boguszów\"_220_110_kV"/RConn3 -- bus212/LConn1
  T_153838553_220000;110000_Stacja_elektroenergetyczna_„Łośnice”_220_110kV/RConn1 -- L_153838553/LConn1
  T_153838553_220000;110000_Stacja_elektroenergetyczna_„Łośnice”_220_110kV/RConn2 -- L_153838553/LConn2
  L_153838553/LConn3 -- T_153838553_220000;110000_Stacja_elektroenergetyczna_„Łośnice”_220_110kV/RConn3 -- bus213/LConn1
  "T_248088256__Stacja_elektroenergetyczna_\"Stalowa_Wola\"_220_110_kV"/RConn1 -- L_248088256/LConn1
  "T_248088256__Stacja_elektroenergetyczna_\"Stalowa_Wola\"_220_110_kV"/RConn2 -- L_248088256/LConn2
  L_248088256/LConn3 -- "T_248088256__Stacja_elektroenergetyczna_\"Stalowa_Wola\"_220_110_kV"/RConn3 -- bus214/LConn1
  "T_191352746_220000;110000_Stacja_elektroenergetyczna_\"Chmielów\"_220_110_kV"/RConn1 -- L_191352746/LConn1
  "T_191352746_220000;110000_Stacja_elektroenergetyczna_\"Chmielów\"_220_110_kV"/RConn2 -- L_191352746/LConn2
  L_191352746/LConn3 -- "T_191352746_220000;110000_Stacja_elektroenergetyczna_\"Chmielów\"_220_110_kV"/RConn3 -- bus215/LConn1
  "T_228154083_220000;110000_Stacja_elektroenergetyczna_\"KIELCE_PIASKI\"_220_110_30_15kV"/RConn1 -- L_228154083/LConn1
  "T_228154083_220000;110000_Stacja_elektroenergetyczna_\"KIELCE_PIASKI\"_220_110_30_15kV"/RConn2 -- L_228154083/LConn2
  L_228154083/LConn3 -- "T_228154083_220000;110000_Stacja_elektroenergetyczna_\"KIELCE_PIASKI\"_220_110_30_15kV"/RConn3 -- bus216/LConn1
  "T_199098055_220000;110000_Stacja_elektroenergetyczna_\"Radkowice\"_220_110_30_15kV"/RConn1 -- L_199098055/LConn1
  "T_199098055_220000;110000_Stacja_elektroenergetyczna_\"Radkowice\"_220_110_30_15kV"/RConn2 -- L_199098055/LConn2
  L_199098055/LConn3 -- "T_199098055_220000;110000_Stacja_elektroenergetyczna_\"Radkowice\"_220_110_30_15kV"/RConn3 -- bus217/LConn1
  T_179279860_220000;110000_Stacja_elektroenergetyczna_„Ząbkowice”_220_110_kV/RConn1 -- L_179279860/LConn1
  T_179279860_220000;110000_Stacja_elektroenergetyczna_„Ząbkowice”_220_110_kV/RConn2 -- L_179279860/LConn2
  L_179279860/LConn3 -- T_179279860_220000;110000_Stacja_elektroenergetyczna_„Ząbkowice”_220_110_kV/RConn3 -- bus218/LConn1
  "T_224727316__Stacja_elektroenergetyczna_\"Huta_Częstochowa\"_220_110_kV"/RConn1 -- L_224727316/LConn1
  "T_224727316__Stacja_elektroenergetyczna_\"Huta_Częstochowa\"_220_110_kV"/RConn2 -- L_224727316/LConn2
  L_224727316/LConn3 -- "T_224727316__Stacja_elektroenergetyczna_\"Huta_Częstochowa\"_220_110_kV"/RConn3 -- bus219/LConn1
  "T_217899005_220000;110000_Stacja_elektroenergetyczna_\"Wrzosowa\"_220_110_kV"/RConn1 -- L_217899005/LConn1
  "T_217899005_220000;110000_Stacja_elektroenergetyczna_\"Wrzosowa\"_220_110_kV"/RConn2 -- L_217899005/LConn2
  L_217899005/LConn3 -- "T_217899005_220000;110000_Stacja_elektroenergetyczna_\"Wrzosowa\"_220_110_kV"/RConn3 -- bus220/LConn1
  T_29098336_220000;110000_Stacja_elektroenergetyczna_„Piaseczno”_220_110_kV/RConn1 -- L_29098336/LConn1
  T_29098336_220000;110000_Stacja_elektroenergetyczna_„Piaseczno”_220_110_kV/RConn2 -- L_29098336/LConn2
  L_29098336/LConn3 -- T_29098336_220000;110000_Stacja_elektroenergetyczna_„Piaseczno”_220_110_kV/RConn3 -- bus221/LConn1
  "T_255293400_220000;110000_Stacja_elektroenergetyczna_\"Bydgoszcz_Zachód\"_220_110_kV"/RConn1 -- L_255293400/LConn1
  "T_255293400_220000;110000_Stacja_elektroenergetyczna_\"Bydgoszcz_Zachód\"_220_110_kV"/RConn2 -- L_255293400/LConn2
  L_255293400/LConn3 -- "T_255293400_220000;110000_Stacja_elektroenergetyczna_\"Bydgoszcz_Zachód\"_220_110_kV"/RConn3 -- bus222/LConn1
  "T_194903381_220000;110000_Stacja_elektroenergetyczna_\"Chełm\"_220_110_kV"/RConn1 -- L_194903381/LConn1
  "T_194903381_220000;110000_Stacja_elektroenergetyczna_\"Chełm\"_220_110_kV"/RConn2 -- L_194903381/LConn2
  L_194903381/LConn3 -- "T_194903381_220000;110000_Stacja_elektroenergetyczna_\"Chełm\"_220_110_kV"/RConn3 -- bus223/LConn1
  T_177493901__/RConn1 -- L_177493901/LConn1
  T_177493901__/RConn2 -- L_177493901/LConn2
  L_177493901/LConn3 -- T_177493901__/RConn3 -- bus224/LConn1
  T_240806770__/RConn1 -- L_240806770/LConn1
  T_240806770__/RConn2 -- L_240806770/LConn2
  L_240806770/LConn3 -- T_240806770__/RConn3 -- bus225/LConn1
  "T_198635989_220000;110000;30000;15000_Stacja_elektroenergetyczna_\"Boguchwała\"_220_110_kV"/RConn1 -- L_198635989/LConn1
  "T_198635989_220000;110000;30000;15000_Stacja_elektroenergetyczna_\"Boguchwała\"_220_110_kV"/RConn2 -- L_198635989/LConn2
  L_198635989/LConn3 -- "T_198635989_220000;110000;30000;15000_Stacja_elektroenergetyczna_\"Boguchwała\"_220_110_kV"/RConn3 -- bus226/LConn1
  "T_255277953_400000;110000_Stacja_elektroenergetyczna_\"Dobrzeń\"_400_110_kV"/RConn1 -- L_255277953/LConn1
  "T_255277953_400000;110000_Stacja_elektroenergetyczna_\"Dobrzeń\"_400_110_kV"/RConn2 -- L_255277953/LConn2
  L_255277953/LConn3 -- "T_255277953_400000;110000_Stacja_elektroenergetyczna_\"Dobrzeń\"_400_110_kV"/RConn3 -- bus227/LConn1
  T_79033485_400000;110000_Stacja_elektroenergetyczna_„Pasikurowice”_400_110_kV/RConn1 -- L_79033485/LConn1
  T_79033485_400000;110000_Stacja_elektroenergetyczna_„Pasikurowice”_400_110_kV/RConn2 -- L_79033485/LConn2
  L_79033485/LConn3 -- T_79033485_400000;110000_Stacja_elektroenergetyczna_„Pasikurowice”_400_110_kV/RConn3 -- bus228/LConn1
  T_171917072_400000;110000_Stacja_elektroenergetyczna_„Trębaczew”_400_110_kV/RConn1 -- L_171917072/LConn1
  T_171917072_400000;110000_Stacja_elektroenergetyczna_„Trębaczew”_400_110_kV/RConn2 -- L_171917072/LConn2
  L_171917072/LConn3 -- T_171917072_400000;110000_Stacja_elektroenergetyczna_„Trębaczew”_400_110_kV/RConn3 -- bus229/LConn1
  T_40946784_400000;110000_Stacja_elektroenergetyczna_„Tucznawa”_400_110_kV/RConn1 -- L_40946784/LConn1
  T_40946784_400000;110000_Stacja_elektroenergetyczna_„Tucznawa”_400_110_kV/RConn2 -- L_40946784/LConn2
  L_40946784/LConn3 -- T_40946784_400000;110000_Stacja_elektroenergetyczna_„Tucznawa”_400_110_kV/RConn3 -- bus230/LConn1
  "T_293489607_400000;110000_Stacja_elektroenergetyczna_\"Rokitnica\"_400_110kV"/RConn1 -- L_293489607/LConn1
  "T_293489607_400000;110000_Stacja_elektroenergetyczna_\"Rokitnica\"_400_110kV"/RConn2 -- L_293489607/LConn2
  L_293489607/LConn3 -- "T_293489607_400000;110000_Stacja_elektroenergetyczna_\"Rokitnica\"_400_110kV"/RConn3 -- bus231/LConn1
  T_254938713_400000;110000_Stacja_elektroenergetyczna_Kromolice_400_110kV/RConn1 -- L_254938713/LConn1
  T_254938713_400000;110000_Stacja_elektroenergetyczna_Kromolice_400_110kV/RConn2 -- L_254938713/LConn2
  L_254938713/LConn3 -- T_254938713_400000;110000_Stacja_elektroenergetyczna_Kromolice_400_110kV/RConn3 -- bus232/LConn1
  T_169979525__/RConn1 -- L_169979525/LConn1
  T_169979525__/RConn2 -- L_169979525/LConn2
  L_169979525/LConn3 -- T_169979525__/RConn3 -- bus233/LConn1
  T_255314292_450000;400000_SwePol_HVDC_Static_Inverter_Plant/RConn1 -- L_255314292/LConn1
  T_255314292_450000;400000_SwePol_HVDC_Static_Inverter_Plant/RConn2 -- L_255314292/LConn2
  L_255314292/LConn3 -- T_255314292_450000;400000_SwePol_HVDC_Static_Inverter_Plant/RConn3 -- bus234/LConn1
  T_169979526__Capacitator_Bank/RConn1 -- L_169979526/LConn1
  T_169979526__Capacitator_Bank/RConn2 -- L_169979526/LConn2
  L_169979526/LConn3 -- T_169979526__Capacitator_Bank/RConn3 -- bus235/LConn1
  T_169979527__Harmonic_Filter/RConn1 -- L_169979527/LConn1
  T_169979527__Harmonic_Filter/RConn2 -- L_169979527/LConn2
  L_169979527/LConn3 -- T_169979527__Harmonic_Filter/RConn3 -- bus236/LConn1
  T_144646702_400000;110000_Stacja_elektroenergetyczna_„Płock”_400_110_kV/RConn1 -- L_144646702/LConn1
  T_144646702_400000;110000_Stacja_elektroenergetyczna_„Płock”_400_110_kV/RConn2 -- L_144646702/LConn2
  L_144646702/LConn3 -- T_144646702_400000;110000_Stacja_elektroenergetyczna_„Płock”_400_110_kV/RConn3 -- bus237/LConn1
  "T_112614319_400000;110000_Stacja_elektroenergetyczna_\"Gdańsk_Błonia\"_400_110_kV"/RConn1 -- L_112614319/LConn1
  "T_112614319_400000;110000_Stacja_elektroenergetyczna_\"Gdańsk_Błonia\"_400_110_kV"/RConn2 -- L_112614319/LConn2
  L_112614319/LConn3 -- "T_112614319_400000;110000_Stacja_elektroenergetyczna_\"Gdańsk_Błonia\"_400_110_kV"/RConn3 -- bus238/LConn1
  "T_154894455_400000;110000_Stacja_elektroenergetyczna_\"Czarna\"_400_110_kV"/RConn1 -- L_154894455/LConn1
  "T_154894455_400000;110000_Stacja_elektroenergetyczna_\"Czarna\"_400_110_kV"/RConn2 -- L_154894455/LConn2
  L_154894455/LConn3 -- "T_154894455_400000;110000_Stacja_elektroenergetyczna_\"Czarna\"_400_110_kV"/RConn3 -- bus239/LConn1
  "T_255293403_400000;110000_Stacja_elektroenergetyczna_\"Ostrów\"_400_110_kV"/RConn1 -- L_255293403/LConn1
  "T_255293403_400000;110000_Stacja_elektroenergetyczna_\"Ostrów\"_400_110_kV"/RConn2 -- L_255293403/LConn2
  L_255293403/LConn3 -- "T_255293403_400000;110000_Stacja_elektroenergetyczna_\"Ostrów\"_400_110_kV"/RConn3 -- bus240/LConn1
  "T_154510504__Stacja_elektroenergetyczna_\"Wrocław\"_400_110kV"/RConn1 -- L_154510504/LConn1
  "T_154510504__Stacja_elektroenergetyczna_\"Wrocław\"_400_110kV"/RConn2 -- L_154510504/LConn2
  L_154510504/LConn3 -- "T_154510504__Stacja_elektroenergetyczna_\"Wrocław\"_400_110kV"/RConn3 -- bus241/LConn1
  T_169979538__Capacitator_Bank/RConn1 -- L_169979538/LConn1
  T_169979538__Capacitator_Bank/RConn2 -- L_169979538/LConn2
  L_169979538/LConn3 -- T_169979538__Capacitator_Bank/RConn3 -- bus242/LConn1
  "T_86494356_400000;110000_Stacja_elektroenergetyczna_\"Żarnowiec\"_400_110_kV"/RConn1 -- L_86494356/LConn1
  "T_86494356_400000;110000_Stacja_elektroenergetyczna_\"Żarnowiec\"_400_110_kV"/RConn2 -- L_86494356/LConn2
  L_86494356/LConn3 -- "T_86494356_400000;110000_Stacja_elektroenergetyczna_\"Żarnowiec\"_400_110_kV"/RConn3 -- bus243/LConn1
  "T_305265212_400000;110000_Stacja_elektrenergetyczna_400_110kV_\"Słupsk_Wierzbięcino\""/RConn1 -- L_305265212/LConn1
  "T_305265212_400000;110000_Stacja_elektrenergetyczna_400_110kV_\"Słupsk_Wierzbięcino\""/RConn2 -- L_305265212/LConn2
  L_305265212/LConn3 -- "T_305265212_400000;110000_Stacja_elektrenergetyczna_400_110kV_\"Słupsk_Wierzbięcino\""/RConn3 -- bus244/LConn1
  "T_365677253_400000;110000_Stacja_elektrenergetyczna_400_110kV_\"Słupsk_Wierzbięcino\""/RConn1 -- L_365677253/LConn1
  "T_365677253_400000;110000_Stacja_elektrenergetyczna_400_110kV_\"Słupsk_Wierzbięcino\""/RConn2 -- L_365677253/LConn2
  L_365677253/LConn3 -- "T_365677253_400000;110000_Stacja_elektrenergetyczna_400_110kV_\"Słupsk_Wierzbięcino\""/RConn3 -- bus245/LConn1
  T_216446549__/RConn1 -- L_216446549/LConn1
  T_216446549__/RConn2 -- L_216446549/LConn2
  L_216446549/LConn3 -- T_216446549__/RConn3 -- bus246/LConn1
  "T_255972397_400000;110000_Stacja_elektroenergetyczna_400_110kV_\"Siedlce_Ujrzanów\""/RConn1 -- L_255972397/LConn1
  "T_255972397_400000;110000_Stacja_elektroenergetyczna_400_110kV_\"Siedlce_Ujrzanów\""/RConn2 -- L_255972397/LConn2
  L_255972397/LConn3 -- "T_255972397_400000;110000_Stacja_elektroenergetyczna_400_110kV_\"Siedlce_Ujrzanów\""/RConn3 -- bus247/LConn1
  "T_255973806_400000_Stacja_elektrenergetyczna_400kV_\"Stanisławów\""/RConn1 -- L_255973806/LConn1
  "T_255973806_400000_Stacja_elektrenergetyczna_400kV_\"Stanisławów\""/RConn2 -- L_255973806/LConn2
  L_255973806/LConn3 -- "T_255973806_400000_Stacja_elektrenergetyczna_400kV_\"Stanisławów\""/RConn3 -- bus248/LConn1
  "T_91384044_400000;110000_Stacja_elektroenergetyczna_\"Mościska\"_400_110_kV"/RConn1 -- L_91384044/LConn1
  "T_91384044_400000;110000_Stacja_elektroenergetyczna_\"Mościska\"_400_110_kV"/RConn2 -- L_91384044/LConn2
  L_91384044/LConn3 -- "T_91384044_400000;110000_Stacja_elektroenergetyczna_\"Mościska\"_400_110_kV"/RConn3 -- bus249/LConn1
  "T_148060965_400000;110000_Stacja_elektroenergetyczna_\"Lublin\"_400_110kV"/RConn1 -- L_148060965/LConn1
  "T_148060965_400000;110000_Stacja_elektroenergetyczna_\"Lublin\"_400_110kV"/RConn2 -- L_148060965/LConn2
  L_148060965/LConn3 -- "T_148060965_400000;110000_Stacja_elektroenergetyczna_\"Lublin\"_400_110kV"/RConn3 -- bus250/LConn1
  "T_303870256_400000_Stacja_elektroenergetyczna_\"Ełk_Bis\"_400_kV"/RConn1 -- L_303870256/LConn1
  "T_303870256_400000_Stacja_elektroenergetyczna_\"Ełk_Bis\"_400_kV"/RConn2 -- L_303870256/LConn2
  L_303870256/LConn3 -- "T_303870256_400000_Stacja_elektroenergetyczna_\"Ełk_Bis\"_400_kV"/RConn3 -- bus251/LConn1
  "T_255972326_400000_Stacja_elektrenergetyczna_400kV_\"Łomża\""/RConn1 -- L_255972326/LConn1
  "T_255972326_400000_Stacja_elektrenergetyczna_400kV_\"Łomża\""/RConn2 -- L_255972326/LConn2
  L_255972326/LConn3 -- "T_255972326_400000_Stacja_elektrenergetyczna_400kV_\"Łomża\""/RConn3 -- bus252/LConn1
  T_293489663_400000;110000_Stacja_elektroenergetyczna_„Narew”_400_110_kV/RConn1 -- L_293489663/LConn1
  T_293489663_400000;110000_Stacja_elektroenergetyczna_„Narew”_400_110_kV/RConn2 -- L_293489663/LConn2
  L_293489663/LConn3 -- T_293489663_400000;110000_Stacja_elektroenergetyczna_„Narew”_400_110_kV/RConn3 -- bus253/LConn1
  "T_166838338_400000;110000_Stacja_elektroenergetyczna_\"Krosno_Iskrzynia\"_400_110_kV"/RConn1 -- L_166838338/LConn1
  "T_166838338_400000;110000_Stacja_elektroenergetyczna_\"Krosno_Iskrzynia\"_400_110_kV"/RConn2 -- L_166838338/LConn2
  L_166838338/LConn3 -- "T_166838338_400000;110000_Stacja_elektroenergetyczna_\"Krosno_Iskrzynia\"_400_110_kV"/RConn3 -- bus254/LConn1
  T_166710856_400000;110000_Stacja_elektroenergetyczna_„Tarnów”_400_110_kV/RConn1 -- L_166710856/LConn1
  T_166710856_400000;110000_Stacja_elektroenergetyczna_„Tarnów”_400_110_kV/RConn2 -- L_166710856/LConn2
  L_166710856/LConn3 -- T_166710856_400000;110000_Stacja_elektroenergetyczna_„Tarnów”_400_110_kV/RConn3 -- bus255/LConn1
  T_215282393_750000;400000;110000_Rzeszów_Systemowa_(Widełka)_750_400_110_kV/RConn1 -- L_215282393/LConn1
  T_215282393_750000;400000;110000_Rzeszów_Systemowa_(Widełka)_750_400_110_kV/RConn2 -- L_215282393/LConn2
  L_215282393/LConn3 -- T_215282393_750000;400000;110000_Rzeszów_Systemowa_(Widełka)_750_400_110_kV/RConn3 -- bus256/LConn1
